simulink model "s_deng_rev1_13_wide"  (R2016b)
(part 3 of 74)

      mask prompts: io_dir "I/O direction"; io_delay "I/O delay"; sample_period "Sample period"; names "Bitfield names [msb...lsb]"; bitwidths "Bitfield widths"; bin_pts "Bitfield binary pts"; arith_types "Bitfield types, ufix=0, fix=1, bool=2"; sim_port "Provide sim input/output?"; show_format "Print format string?"
      mask help: A 32-bit software-accessible register. Can be divided into bitfields of varying widths and types using the fields in the block mask.
      mask init:
      | swreg_init(gcb)
      settings: AttributesFormatString=1input:uf32.0 = 32 bits
      mask TypeOptions io_dir: To Processor | From Processor
      mask Callback io_dir:
      | mask_enables = get_param(gcb, 'MaskEnables');
      | mask_names = get_param(gcb, 'MaskNames');
      | if strcmp(get_param(gcb, 'io_dir'), 'To Processor'),
      |     mask_enables{ismember(mask_names, 'sample_period')} = 'off';
      | else
      |     mask_enables{ismember(mask_names, 'sample_period')} = 'on';
      | end
      | set_param(gcb, 'MaskEnables', mask_enables);
  rpt_length_wng0 : Subsystem  Tag=xps:sw_reg  AncestorBlock=xps_library/software_register  mask(swreg){io_dir=From Processor, io_delay=1, sample_period=1, names=samples, bitwidths=32, bin_pts=0, arith_types=0, sim_port=on, show_format=on}
      mask prompts: io_dir "I/O direction"; io_delay "I/O delay"; sample_period "Sample period"; names "Bitfield names [msb...lsb]"; bitwidths "Bitfield widths"; bin_pts "Bitfield binary pts"; arith_types "Bitfield types, ufix=0, fix=1, bool=2"; sim_port "Provide sim input/output?"; show_format "Print format string?"
      mask help: A 32-bit software-accessible register. Can be divided into bitfields of varying widths and types using the fields in the block mask.
      mask init:
      | swreg_init(gcb)
      settings: AttributesFormatString=1input:uf32.0 = 32 bits
      mask TypeOptions io_dir: To Processor | From Processor
      mask Callback io_dir:
      | mask_enables = get_param(gcb, 'MaskEnables');
      | mask_names = get_param(gcb, 'MaskNames');
      | if strcmp(get_param(gcb, 'io_dir'), 'To Processor'),
      |     mask_enables{ismember(mask_names, 'sample_period')} = 'off';
      | else
      |     mask_enables{ismember(mask_names, 'sample_period')} = 'on';
      | end
      | set_param(gcb, 'MaskEnables', mask_enables);
  rpt_load_time_lsw_wng0 : Subsystem  Tag=xps:sw_reg  AncestorBlock=xps_library/software_register  mask(swreg){io_dir=From Processor, io_delay=1, sample_period=1, names=reg, bitwidths=32, bin_pts=0, arith_types=0, sim_port=on, show_format=on}
      mask prompts: io_dir "I/O direction"; io_delay "I/O delay"; sample_period "Sample period"; names "Bitfield names [msb...lsb]"; bitwidths "Bitfield widths"; bin_pts "Bitfield binary pts"; arith_types "Bitfield types, ufix=0, fix=1, bool=2"; sim_port "Provide sim input/output?"; show_format "Print format string?"
      mask help: A 32-bit software-accessible register. Can be divided into bitfields of varying widths and types using the fields in the block mask.
      mask init:
      | swreg_init(gcb)
      settings: AttributesFormatString=1input:uf32.0 = 32 bits
      mask TypeOptions io_dir: To Processor | From Processor
      mask Callback io_dir:
      | mask_enables = get_param(gcb, 'MaskEnables');
      | mask_names = get_param(gcb, 'MaskNames');
      | if strcmp(get_param(gcb, 'io_dir'), 'To Processor'),
      |     mask_enables{ismember(mask_names, 'sample_period')} = 'off';
      | else
      |     mask_enables{ismember(mask_names, 'sample_period')} = 'on';
      | end
      | set_param(gcb, 'MaskEnables', mask_enables);
  rpt_load_time_msw_wng0 : Subsystem  Tag=xps:sw_reg  AncestorBlock=xps_library/software_register  mask(swreg){io_dir=From Processor, io_delay=1, sample_period=1, names=reg, bitwidths=32, bin_pts=0, arith_types=0, sim_port=on, show_format=on}
      mask prompts: io_dir "I/O direction"; io_delay "I/O delay"; sample_period "Sample period"; names "Bitfield names [msb...lsb]"; bitwidths "Bitfield widths"; bin_pts "Bitfield binary pts"; arith_types "Bitfield types, ufix=0, fix=1, bool=2"; sim_port "Provide sim input/output?"; show_format "Print format string?"
      mask help: A 32-bit software-accessible register. Can be divided into bitfields of varying widths and types using the fields in the block mask.
      mask init:
      | swreg_init(gcb)
      settings: AttributesFormatString=1input:uf32.0 = 32 bits
      mask TypeOptions io_dir: To Processor | From Processor
      mask Callback io_dir:
      | mask_enables = get_param(gcb, 'MaskEnables');
      | mask_names = get_param(gcb, 'MaskNames');
      | if strcmp(get_param(gcb, 'io_dir'), 'To Processor'),
      |     mask_enables{ismember(mask_names, 'sample_period')} = 'off';
      | else
      |     mask_enables{ismember(mask_names, 'sample_period')} = 'on';
      | end
      | set_param(gcb, 'MaskEnables', mask_enables);
  sample_masking : Subsystem  mask{dbwidth=1}
      mask prompts: dbwidth "Data bitwidth:"
  scale_cwg0 : Subsystem  Tag=xps:sw_reg  AncestorBlock=xps_library/software_register  mask(swreg){io_dir=From Processor, io_delay=1, sample_period=1, names=[scale dummy], bitwidths=16, bin_pts=15, arith_types=0, sim_port=on, show_format=on}
      mask prompts: io_dir "I/O direction"; io_delay "I/O delay"; sample_period "Sample period"; names "Bitfield names [msb...lsb]"; bitwidths "Bitfield widths"; bin_pts "Bitfield binary pts"; arith_types "Bitfield types, ufix=0, fix=1, bool=2"; sim_port "Provide sim input/output?"; show_format "Print format string?"
      mask help: A 32-bit software-accessible register. Can be divided into bitfields of varying widths and types using the fields in the block mask.
      mask init:
      | swreg_init(gcb)
      settings: AttributesFormatString=2 inputs:uf16.15,uf16.15 = 32 bits
      mask TypeOptions io_dir: To Processor | From Processor
      mask Callback io_dir:
      | mask_enables = get_param(gcb, 'MaskEnables');
      | mask_names = get_param(gcb, 'MaskNames');
      | if strcmp(get_param(gcb, 'io_dir'), 'To Processor'),
      |     mask_enables{ismember(mask_names, 'sample_period')} = 'off';
      | else
      |     mask_enables{ismember(mask_names, 'sample_period')} = 'on';
      | end
      | set_param(gcb, 'MaskEnables', mask_enables);
  scale_cwg1 : Subsystem  Tag=xps:sw_reg  AncestorBlock=xps_library/software_register  mask(swreg){io_dir=From Processor, io_delay=1, sample_period=1, names=[scale dummy], bitwidths=16, bin_pts=15, arith_types=0, sim_port=on, show_format=on}
      mask prompts: io_dir "I/O direction"; io_delay "I/O delay"; sample_period "Sample period"; names "Bitfield names [msb...lsb]"; bitwidths "Bitfield widths"; bin_pts "Bitfield binary pts"; arith_types "Bitfield types, ufix=0, fix=1, bool=2"; sim_port "Provide sim input/output?"; show_format "Print format string?"
      mask help: A 32-bit software-accessible register. Can be divided into bitfields of varying widths and types using the fields in the block mask.
      mask init:
      | swreg_init(gcb)
      settings: AttributesFormatString=2 inputs:uf16.15,uf16.15 = 32 bits
      mask TypeOptions io_dir: To Processor | From Processor
      mask Callback io_dir:
      | mask_enables = get_param(gcb, 'MaskEnables');
      | mask_names = get_param(gcb, 'MaskNames');
      | if strcmp(get_param(gcb, 'io_dir'), 'To Processor'),
      |     mask_enables{ismember(mask_names, 'sample_period')} = 'off';
      | else
      |     mask_enables{ismember(mask_names, 'sample_period')} = 'on';
      | end
      | set_param(gcb, 'MaskEnables', mask_enables);
  scale_cwg_corr : Subsystem  Tag=xps:sw_reg  AncestorBlock=xps_library/software_register  mask(swreg){io_dir=From Processor, io_delay=1, sample_period=1, names=[scale dummy], bitwidths=16, bin_pts=15, arith_types=0, sim_port=on, show_format=on}
      mask prompts: io_dir "I/O direction"; io_delay "I/O delay"; sample_period "Sample period"; names "Bitfield names [msb...lsb]"; bitwidths "Bitfield widths"; bin_pts "Bitfield binary pts"; arith_types "Bitfield types, ufix=0, fix=1, bool=2"; sim_port "Provide sim input/output?"; show_format "Print format string?"
      mask help: A 32-bit software-accessible register. Can be divided into bitfields of varying widths and types using the fields in the block mask.
      mask init:
      | swreg_init(gcb)
      settings: AttributesFormatString=2 inputs:uf16.15,uf16.15 = 32 bits
      mask TypeOptions io_dir: To Processor | From Processor
      mask Callback io_dir:
      | mask_enables = get_param(gcb, 'MaskEnables');
      | mask_names = get_param(gcb, 'MaskNames');
      | if strcmp(get_param(gcb, 'io_dir'), 'To Processor'),
      |     mask_enables{ismember(mask_names, 'sample_period')} = 'off';
      | else
      |     mask_enables{ismember(mask_names, 'sample_period')} = 'on';
      | end
      | set_param(gcb, 'MaskEnables', mask_enables);
  scale_out0 : Subsystem  Tag=xps:sw_reg  AncestorBlock=xps_library/software_register  mask(swreg){io_dir=From Processor, io_delay=1, sample_period=1, names=[scale dummy], bitwidths=16, bin_pts=15, arith_types=0, sim_port=on, show_format=on}
      mask prompts: io_dir "I/O direction"; io_delay "I/O delay"; sample_period "Sample period"; names "Bitfield names [msb...lsb]"; bitwidths "Bitfield widths"; bin_pts "Bitfield binary pts"; arith_types "Bitfield types, ufix=0, fix=1, bool=2"; sim_port "Provide sim input/output?"; show_format "Print format string?"
      mask help: A 32-bit software-accessible register. Can be divided into bitfields of varying widths and types using the fields in the block mask.
      mask init:
      | swreg_init(gcb)
      settings: AttributesFormatString=2 inputs:uf16.15,uf16.15 = 32 bits
      mask TypeOptions io_dir: To Processor | From Processor
      mask Callback io_dir:
      | mask_enables = get_param(gcb, 'MaskEnables');
      | mask_names = get_param(gcb, 'MaskNames');
      | if strcmp(get_param(gcb, 'io_dir'), 'To Processor'),
      |     mask_enables{ismember(mask_names, 'sample_period')} = 'off';
      | else
      |     mask_enables{ismember(mask_names, 'sample_period')} = 'on';
      | end
      | set_param(gcb, 'MaskEnables', mask_enables);
  scale_out1 : Subsystem  Tag=xps:sw_reg  AncestorBlock=xps_library/software_register  mask(swreg){io_dir=From Processor, io_delay=1, sample_period=1, names=[scale dummy], bitwidths=16, bin_pts=15, arith_types=0, sim_port=on, show_format=on}
      mask prompts: io_dir "I/O direction"; io_delay "I/O delay"; sample_period "Sample period"; names "Bitfield names [msb...lsb]"; bitwidths "Bitfield widths"; bin_pts "Bitfield binary pts"; arith_types "Bitfield types, ufix=0, fix=1, bool=2"; sim_port "Provide sim input/output?"; show_format "Print format string?"
      mask help: A 32-bit software-accessible register. Can be divided into bitfields of varying widths and types using the fields in the block mask.
      mask init:
      | swreg_init(gcb)
      settings: AttributesFormatString=2 inputs:uf16.15,uf16.15 = 32 bits
      mask TypeOptions io_dir: To Processor | From Processor
      mask Callback io_dir:
      | mask_enables = get_param(gcb, 'MaskEnables');
      | mask_names = get_param(gcb, 'MaskNames');
      | if strcmp(get_param(gcb, 'io_dir'), 'To Processor'),
      |     mask_enables{ismember(mask_names, 'sample_period')} = 'off';
      | else
      |     mask_enables{ismember(mask_names, 'sample_period')} = 'on';
      | end
      | set_param(gcb, 'MaskEnables', mask_enables);
  scale_wng0 : Subsystem  Tag=xps:sw_reg  AncestorBlock=xps_library/software_register  mask(swreg){io_dir=From Processor, io_delay=1, sample_period=1, names=[scale dummy], bitwidths=16, bin_pts=15, arith_types=0, sim_port=on, show_format=on}
      mask prompts: io_dir "I/O direction"; io_delay "I/O delay"; sample_period "Sample period"; names "Bitfield names [msb...lsb]"; bitwidths "Bitfield widths"; bin_pts "Bitfield binary pts"; arith_types "Bitfield types, ufix=0, fix=1, bool=2"; sim_port "Provide sim input/output?"; show_format "Print format string?"
      mask help: A 32-bit software-accessible register. Can be divided into bitfields of varying widths and types using the fields in the block mask.
      mask init:
      | swreg_init(gcb)
      settings: AttributesFormatString=2 inputs:uf16.15,uf16.15 = 32 bits
      mask TypeOptions io_dir: To Processor | From Processor
      mask Callback io_dir:
      | mask_enables = get_param(gcb, 'MaskEnables');
      | mask_names = get_param(gcb, 'MaskNames');
      | if strcmp(get_param(gcb, 'io_dir'), 'To Processor'),
      |     mask_enables{ismember(mask_names, 'sample_period')} = 'off';
      | else
      |     mask_enables{ismember(mask_names, 'sample_period')} = 'on';
      | end
      | set_param(gcb, 'MaskEnables', mask_enables);
  scale_wng1 : Subsystem  Tag=xps:sw_reg  AncestorBlock=xps_library/software_register  mask(swreg){io_dir=From Processor, io_delay=1, sample_period=1, names=[scale dummy], bitwidths=16, bin_pts=15, arith_types=0, sim_port=on, show_format=on}
      mask prompts: io_dir "I/O direction"; io_delay "I/O delay"; sample_period "Sample period"; names "Bitfield names [msb...lsb]"; bitwidths "Bitfield widths"; bin_pts "Bitfield binary pts"; arith_types "Bitfield types, ufix=0, fix=1, bool=2"; sim_port "Provide sim input/output?"; show_format "Print format string?"
      mask help: A 32-bit software-accessible register. Can be divided into bitfields of varying widths and types using the fields in the block mask.
      mask init:
      | swreg_init(gcb)
      settings: AttributesFormatString=2 inputs:uf16.15,uf16.15 = 32 bits
      mask TypeOptions io_dir: To Processor | From Processor
      mask Callback io_dir:
      | mask_enables = get_param(gcb, 'MaskEnables');
      | mask_names = get_param(gcb, 'MaskNames');
      | if strcmp(get_param(gcb, 'io_dir'), 'To Processor'),
      |     mask_enables{ismember(mask_names, 'sample_period')} = 'off';
      | else
      |     mask_enables{ismember(mask_names, 'sample_period')} = 'on';
      | end
      | set_param(gcb, 'MaskEnables', mask_enables);
  scale_wng_corr : Subsystem  Tag=xps:sw_reg  AncestorBlock=xps_library/software_register  mask(swreg){io_dir=From Processor, io_delay=1, sample_period=1, names=[scale dummy], bitwidths=16, bin_pts=15, arith_types=0, sim_port=on, show_format=on}
      mask prompts: io_dir "I/O direction"; io_delay "I/O delay"; sample_period "Sample period"; names "Bitfield names [msb...lsb]"; bitwidths "Bitfield widths"; bin_pts "Bitfield binary pts"; arith_types "Bitfield types, ufix=0, fix=1, bool=2"; sim_port "Provide sim input/output?"; show_format "Print format string?"
      mask help: A 32-bit software-accessible register. Can be divided into bitfields of varying widths and types using the fields in the block mask.
      mask init:
      | swreg_init(gcb)
      settings: AttributesFormatString=2 inputs:uf16.15,uf16.15 = 32 bits
      mask TypeOptions io_dir: To Processor | From Processor
      mask Callback io_dir:
      | mask_enables = get_param(gcb, 'MaskEnables');
      | mask_names = get_param(gcb, 'MaskNames');
      | if strcmp(get_param(gcb, 'io_dir'), 'To Processor'),
      |     mask_enables{ismember(mask_names, 'sample_period')} = 'off';
      | else
      |     mask_enables{ismember(mask_names, 'sample_period')} = 'on';
      | end
      | set_param(gcb, 'MaskEnables', mask_enables);
  slice1 : xbsIndex_r4/Slice  nbits=32  boolean_output=off  mode=Lower Bit Location + Width  bit1=-7  base1=MSB of Input  bit0=0  base0=LSB of Input  dbl_ovrd=off  block_type=slice
  slice2 : xbsIndex_r4/Slice  nbits=32  boolean_output=off  mode=Lower Bit Location + Width  bit1=-32  base1=MSB of Input  bit0=32  base0=LSB of Input  dbl_ovrd=off  block_type=slice
  spead_detail : Subsystem  Tag=casper:bitsnap  AncestorBlock=casper_library_scopes/bitfield_snapshot  mask(bitsnap){io_names=[eof we], io_widths=[1 1], io_bps=[0 0], io_types=[2 2], show_format=on, snap_storage=bram, snap_dram_dimm=2, snap_dram_clock=250, snap_nsamples=15, snap_data_width=32, snap_offset=off, snap_circap=off, snap_value=off, snap_ext_arm=off, snap_provide_outputs=on, snap_use_dsp48=on, snap_delay=2, extra_names=[c d], extra_widths=[30 2], extra_bps=[0 0], extra_types=[0 0]}
      mask prompts: io_names "Names [msb...lsb]"; io_widths "Bitwidths [msb...lsb]"; io_bps "Binary pts [msb...lsb]"; io_types "Data types [msb...lsb], ufix=0, fix=1, bool=2"; show_format "Print format string?"; snap_storage "Storage medium"; snap_dram_dimm "DRAM dimm"; snap_dram_clock "DRAM clock rate"; snap_nsamples "Number of Samples (2^?)"; snap_data_width "Data width"; snap_offset "Start delay support"; snap_circap "Circular capture support"; snap_value "Extra value capture support"; snap_ext_arm "External arm support"; snap_provide_outputs "Provide outputs"; snap_use_dsp48 "Use DSP48s to implement counters"; snap_delay "Pre-snapshot delay"; extra_names "Names [msb...lsb]"; extra_widths "Widths [msb...lsb]"; extra_bps "Binary pts [msb...lsb]"; extra_types "Data types [msb...lsb], ufix=0, fix=1, bool=2"
      mask help:
      | A wrapped snapshot block. Allows specification of inputs to a snapblock word so the toolflow can automatically set up the scope.
      | See documentation for snapshot for explanation of parameters.
      mask init:
      | bitsnap_init(gcb);
      settings: AttributesFormatString=|
      | snap(2):b,b = 2 bits\n32 wide, 32768 deep
      | debugID: 29988897
      mask TypeOptions snap_storage: bram | dram
      mask Callback snap_storage: bitsnap_callback();
      mask TypeOptions snap_dram_dimm: 1 | 2 | 3 | 4
      mask TypeOptions snap_dram_clock: 200 | 250 | 266 | 300 | 333
      mask TypeOptions snap_data_width: 8 | 16 | 32 | 64 | 128
      mask Callback snap_value: bitsnap_callback();
      mask Callback snap_ext_arm: bitsnap_callback();
      mask Callback snap_provide_outputs: bitsnap_callback();
  spead_pack0 : Subsystem  Tag=casper:spead_pack  AncestorBlock=casper_library_communications/spead_pack  mask(pkt_pack_mask){max_pkt_len_bits=10, header_ids=0x1600, 0x3101, 0x3102, header_ind_ids=0x3300, spead_msw=64, spead_lsw=48, spead_version=4, bytes_per_word=8}
      mask prompts: max_pkt_len_bits "Max pkt length, 2^? 64-bit words"; header_ids "SPEAD direct address IDs (decimal)"; header_ind_ids "SPEAD indirect address IDs (decimal)"; spead_msw "SPEAD Flavour (MSw)"; spead_lsw "SPEAD Flavour (LSw)"; spead_version "SPEAD version"; bytes_per_word "Word size, in bytes"
      mask help:
      | This block generates SPEAD-compliant packets from a datastream.
      |
      | Packets are created with a fixed header followed by a number of 64-bit items.
      |
      | Requires a 64-bit data stream.
      |
      | The data_ready signal is one cycle BEFORE valid data! Does not have to be with a valid signal either.
      mask init:
      | if floor(log2(bytes_per_word)) ~= log2(bytes_per_word)
      |     error('Bytes per word should be a power of two.');
      | end
      | 
      | spead_pack_init(gcb)
  spead_pack1 : Subsystem  Tag=casper:spead_pack  AncestorBlock=casper_library_communications/spead_pack  mask(pkt_pack_mask){max_pkt_len_bits=10, header_ids=0x1600, 0x3101, 0x3102, header_ind_ids=0x3300, spead_msw=64, spead_lsw=48, spead_version=4, bytes_per_word=8}
      mask prompts: max_pkt_len_bits "Max pkt length, 2^? 64-bit words"; header_ids "SPEAD direct address IDs (decimal)"; header_ind_ids "SPEAD indirect address IDs (decimal)"; spead_msw "SPEAD Flavour (MSw)"; spead_lsw "SPEAD Flavour (LSw)"; spead_version "SPEAD version"; bytes_per_word "Word size, in bytes"
      mask help:
      | This block generates SPEAD-compliant packets from a datastream.
      |
      | Packets are created with a fixed header followed by a number of 64-bit items.
      |
      | Requires a 64-bit data stream.
      |
      | The data_ready signal is one cycle BEFORE valid data! Does not have to be with a valid signal either.
      mask init:
      | if floor(log2(bytes_per_word)) ~= log2(bytes_per_word)
      |     error('Bytes per word should be a power of two.');
      | end
      | 
      | spead_pack_init(gcb)
  spead_pack2 : Subsystem  Tag=casper:spead_pack  AncestorBlock=casper_library_communications/spead_pack  mask(pkt_pack_mask){max_pkt_len_bits=10, header_ids=0x1600, 0x3101, 0x3102, header_ind_ids=0x3300, spead_msw=64, spead_lsw=48, spead_version=4, bytes_per_word=8}
      mask prompts: max_pkt_len_bits "Max pkt length, 2^? 64-bit words"; header_ids "SPEAD direct address IDs (decimal)"; header_ind_ids "SPEAD indirect address IDs (decimal)"; spead_msw "SPEAD Flavour (MSw)"; spead_lsw "SPEAD Flavour (LSw)"; spead_version "SPEAD version"; bytes_per_word "Word size, in bytes"
      mask help:
      | This block generates SPEAD-compliant packets from a datastream.
      |
      | Packets are created with a fixed header followed by a number of 64-bit items.
      |
      | Requires a 64-bit data stream.
      |
      | The data_ready signal is one cycle BEFORE valid data! Does not have to be with a valid signal either.
      mask init:
      | if floor(log2(bytes_per_word)) ~= log2(bytes_per_word)
      |     error('Bytes per word should be a power of two.');
      | end
      | 
      | spead_pack_init(gcb)
  spead_pack3 : Subsystem  Tag=casper:spead_pack  AncestorBlock=casper_library_communications/spead_pack  mask(pkt_pack_mask){max_pkt_len_bits=10, header_ids=0x1600, 0x3101, 0x3102, header_ind_ids=0x3300, spead_msw=64, spead_lsw=48, spead_version=4, bytes_per_word=8}
      mask prompts: max_pkt_len_bits "Max pkt length, 2^? 64-bit words"; header_ids "SPEAD direct address IDs (decimal)"; header_ind_ids "SPEAD indirect address IDs (decimal)"; spead_msw "SPEAD Flavour (MSw)"; spead_lsw "SPEAD Flavour (LSw)"; spead_version "SPEAD version"; bytes_per_word "Word size, in bytes"
      mask help:
      | This block generates SPEAD-compliant packets from a datastream.
      |
      | Packets are created with a fixed header followed by a number of 64-bit items.
      |
      | Requires a 64-bit data stream.
      |
      | The data_ready signal is one cycle BEFORE valid data! Does not have to be with a valid signal either.
      mask init:
      | if floor(log2(bytes_per_word)) ~= log2(bytes_per_word)
      |     error('Bytes per word should be a power of two.');
      | end
      | 
      | spead_pack_init(gcb)
  spead_snap0 : Subsystem  Tag=casper:bitsnap  AncestorBlock=casper_library_scopes/bitfield_snapshot  mask(bitsnap){io_names=[d64], io_widths=64, io_bps=0, io_types=0, show_format=on, snap_storage=bram, snap_dram_dimm=2, snap_dram_clock=250, snap_nsamples=15, snap_data_width=64, snap_offset=off, snap_circap=off, snap_value=off, snap_ext_arm=off, snap_provide_outputs=on, snap_use_dsp48=on, snap_delay=2, extra_names=[c d], extra_widths=[30 2], extra_bps=[0 0], extra_types=[0 0]}
      mask prompts: io_names "Names [msb...lsb]"; io_widths "Bitwidths [msb...lsb]"; io_bps "Binary pts [msb...lsb]"; io_types "Data types [msb...lsb], ufix=0, fix=1, bool=2"; show_format "Print format string?"; snap_storage "Storage medium"; snap_dram_dimm "DRAM dimm"; snap_dram_clock "DRAM clock rate"; snap_nsamples "Number of Samples (2^?)"; snap_data_width "Data width"; snap_offset "Start delay support"; snap_circap "Circular capture support"; snap_value "Extra value capture support"; snap_ext_arm "External arm support"; snap_provide_outputs "Provide outputs"; snap_use_dsp48 "Use DSP48s to implement counters"; snap_delay "Pre-snapshot delay"; extra_names "Names [msb...lsb]"; extra_widths "Widths [msb...lsb]"; extra_bps "Binary pts [msb...lsb]"; extra_types "Data types [msb...lsb], ufix=0, fix=1, bool=2"
      mask help:
      | A wrapped snapshot block. Allows specification of inputs to a snapblock word so the toolflow can automatically set up the scope.
      | See documentation for snapshot for explanation of parameters.
      mask init:
      | bitsnap_init(gcb);
      settings: AttributesFormatString=|
      | snap(1):uf64.0 = 64 bits\n64 wide, 32768 deep
      | debugID: 109311942
      mask TypeOptions snap_storage: bram | dram
      mask Callback snap_storage: bitsnap_callback();
      mask TypeOptions snap_dram_dimm: 1 | 2 | 3 | 4
      mask TypeOptions snap_dram_clock: 200 | 250 | 266 | 300 | 333
      mask TypeOptions snap_data_width: 8 | 16 | 32 | 64 | 128
      mask Callback snap_value: bitsnap_callback();
      mask Callback snap_ext_arm: bitsnap_callback();
      mask Callback snap_provide_outputs: bitsnap_callback();
  speadsnap_control : Subsystem  Tag=xps:sw_reg  AncestorBlock=xps_library/software_register  mask(swreg){io_dir=From Processor, io_delay=0, sample_period=1, names=[speadsnap_arm], bitwidths=1, bin_pts=0, arith_types=2, sim_port=off, show_format=on}
      mask prompts: io_dir "I/O direction"; io_delay "I/O delay"; sample_period "Sample period"; names "Bitfield names [msb...lsb]"; bitwidths "Bitfield widths"; bin_pts "Bitfield binary pts"; arith_types "Bitfield types, ufix=0, fix=1, bool=2"; sim_port "Provide sim input/output?"; show_format "Print format string?"
      mask help: A 32-bit software-accessible register. Can be divided into bitfields of varying widths and types using the fields in the block mask.
      mask init:
      | swreg_init(gcb)
      settings: AttributesFormatString=1input:b = 1 bits
      mask TypeOptions io_dir: To Processor | From Processor
      mask Callback io_dir:
      | mask_enables = get_param(gcb, 'MaskEnables');
      | mask_names = get_param(gcb, 'MaskNames');
      | if strcmp(get_param(gcb, 'io_dir'), 'To Processor'),
      |     mask_enables{ismember(mask_names, 'sample_period')} = 'off';
      | else
      |     mask_enables{ismember(mask_names, 'sample_period')} = 'on';
      | end
      | set_param(gcb, 'MaskEnables', mask_enables);
  speadtime0_offset : Subsystem  Tag=xps:sw_reg  AncestorBlock=xps_library/software_register  mask(swreg){io_dir=From Processor, io_delay=1, sample_period=1, names=speadtime_offset0, bitwidths=32, bin_pts=0, arith_types=0, sim_port=on, show_format=on}
      mask prompts: io_dir "I/O direction"; io_delay "I/O delay"; sample_period "Sample period"; names "Bitfield names [msb...lsb]"; bitwidths "Bitfield widths"; bin_pts "Bitfield binary pts"; arith_types "Bitfield types, ufix=0, fix=1, bool=2"; sim_port "Provide sim input/output?"; show_format "Print format string?"
      mask help: A 32-bit software-accessible register. Can be divided into bitfields of varying widths and types using the fields in the block mask.
      mask init:
      | swreg_init(gcb)
      settings: AttributesFormatString=1input:uf32.0 = 32 bits
      mask TypeOptions io_dir: To Processor | From Processor
      mask Callback io_dir:
      | mask_enables = get_param(gcb, 'MaskEnables');
      | mask_names = get_param(gcb, 'MaskNames');
      | if strcmp(get_param(gcb, 'io_dir'), 'To Processor'),
      |     mask_enables{ismember(mask_names, 'sample_period')} = 'off';
      | else
      |     mask_enables{ismember(mask_names, 'sample_period')} = 'on';
      | end
      | set_param(gcb, 'MaskEnables', mask_enables);
  speadtime1_offset : Subsystem  Tag=xps:sw_reg  AncestorBlock=xps_library/software_register  mask(swreg){io_dir=From Processor, io_delay=1, sample_period=1, names=speadtime_offset1, bitwidths=32, bin_pts=0, arith_types=0, sim_port=on, show_format=on}
      mask prompts: io_dir "I/O direction"; io_delay "I/O delay"; sample_period "Sample period"; names "Bitfield names [msb...lsb]"; bitwidths "Bitfield widths"; bin_pts "Bitfield binary pts"; arith_types "Bitfield types, ufix=0, fix=1, bool=2"; sim_port "Provide sim input/output?"; show_format "Print format string?"
      mask help: A 32-bit software-accessible register. Can be divided into bitfields of varying widths and types using the fields in the block mask.
      mask init:
      | swreg_init(gcb)
      settings: AttributesFormatString=1input:uf32.0 = 32 bits
      mask TypeOptions io_dir: To Processor | From Processor
      mask Callback io_dir:
      | mask_enables = get_param(gcb, 'MaskEnables');
      | mask_names = get_param(gcb, 'MaskNames');
      | if strcmp(get_param(gcb, 'io_dir'), 'To Processor'),
      |     mask_enables{ismember(mask_names, 'sample_period')} = 'off';
      | else
      |     mask_enables{ismember(mask_names, 'sample_period')} = 'on';
      | end
      | set_param(gcb, 'MaskEnables', mask_enables);
  src_sel_cntrl : Subsystem  Tag=xps:sw_reg  AncestorBlock=xps_library/software_register  mask(swreg){io_dir=From Processor, io_delay=1, sample_period=1, names=[src_sel_0 src_sel_1], bitwidths=[2 2], bin_pts=[0 0], arith_types=[0 0], sim_port=on, show_format=on}
      mask prompts: io_dir "I/O direction"; io_delay "I/O delay"; sample_period "Sample period"; names "Bitfield names [msb...lsb]"; bitwidths "Bitfield widths"; bin_pts "Bitfield binary pts"; arith_types "Bitfield types, ufix=0, fix=1, bool=2"; sim_port "Provide sim input/output?"; show_format "Print format string?"
      mask help: A 32-bit software-accessible register. Can be divided into bitfields of varying widths and types using the fields in the block mask.
      mask init:
      | swreg_init(gcb)
      settings: AttributesFormatString=2 inputs:uf2.0,uf2.0 = 4 bits
      mask TypeOptions io_dir: To Processor | From Processor
      mask Callback io_dir:
      | mask_enables = get_param(gcb, 'MaskEnables');
      | mask_names = get_param(gcb, 'MaskNames');
      | if strcmp(get_param(gcb, 'io_dir'), 'To Processor'),
      |     mask_enables{ismember(mask_names, 'sample_period')} = 'off';
      | else
      |     mask_enables{ismember(mask_names, 'sample_period')} = 'on';
      | end
      | set_param(gcb, 'MaskEnables', mask_enables);
  ss_cwg0 : Subsystem  Tag=casper:bitsnap  AncestorBlock=casper_library_scopes/bitfield snapshot  mask(bitsnap){io_names=[d0 d1 d2 d3 d4 d5 d6 d7 gpio_trig], io_widths=[10 10 10 10 10 10 10 10 1], io_bps=[9 9 9 9 9 9 9 9 0], io_types=[1 1 1 1 1 1 1 1 2], show_format=on, snap_storage=bram, snap_dram_dimm=2, snap_dram_clock=250, snap_nsamples=11, snap_data_width=128, snap_offset=on, snap_circap=off, snap_value=off, snap_use_dsp48=off, snap_delay=1, extra_names=[c d], extra_widths=[30 2], extra_bps=[0 0], extra_types=[0 0]}
      mask prompts: io_names "Names [msb...lsb]"; io_widths "Bitwidths [msb...lsb]"; io_bps "Binary pts [msb...lsb]"; io_types "Data types [msb...lsb], ufix=0, fix=1, bool=2"; show_format "Print format string?"; snap_storage "Storage medium"; snap_dram_dimm "DRAM dimm"; snap_dram_clock "DRAM clock rate"; snap_nsamples "Number of Samples (2^?)"; snap_data_width "Data width"; snap_offset "Start delay support"; snap_circap "Circular capture support"; snap_value "Extra value capture support"; snap_use_dsp48 "Use DSP48s to implement counters"; snap_delay "Pre-snapshot delay"; extra_names "Names [msb...lsb]"; extra_widths "Widths [msb...lsb]"; extra_bps "Binary pts [msb...lsb]"; extra_types "Data types [msb...lsb], ufix=0, fix=1, bool=2"
      mask help:
      | A wrapped snapshot block. Allows specification of inputs to a snapblock word so the toolflow can automatically set up the scope.
      | See documentation for snapshot for explanation of parameters.
      mask init:
      | bitsnap_init(gcb);
      settings: AttributesFormatString=|
      | snap(9):f10.9,f10.9,f10.9,f10.9,f10.9,f10.9,f10.9,f10.9,b = 81 bits\n128 wide, 2048 deep
      | debugID: 35994012
      mask TypeOptions snap_storage: bram | dram
      mask Callback snap_storage: bitsnap_callback();
      mask TypeOptions snap_dram_dimm: 1 | 2 | 3 | 4
      mask TypeOptions snap_dram_clock: 200 | 250 | 266 | 300 | 333
      mask TypeOptions snap_data_width: 8 | 16 | 32 | 64 | 128
      mask Callback snap_value: bitsnap_callback();
  ss_cwg1 : Subsystem  Tag=casper:bitsnap  AncestorBlock=casper_library_scopes/bitfield snapshot  mask(bitsnap){io_names=[d0 d1 d2 d3 d4 d5 d6 d7 gpio_trig], io_widths=[10 10 10 10 10 10 10 10 1], io_bps=[9 9 9 9 9 9 9 9 0], io_types=[1 1 1 1 1 1 1 1 2], show_format=on, snap_storage=bram, snap_dram_dimm=2, snap_dram_clock=250, snap_nsamples=11, snap_data_width=128, snap_offset=on, snap_circap=off, snap_value=off, snap_use_dsp48=off, snap_delay=1, extra_names=[c d], extra_widths=[30 2], extra_bps=[0 0], extra_types=[0 0]}
      mask prompts: io_names "Names [msb...lsb]"; io_widths "Bitwidths [msb...lsb]"; io_bps "Binary pts [msb...lsb]"; io_types "Data types [msb...lsb], ufix=0, fix=1, bool=2"; show_format "Print format string?"; snap_storage "Storage medium"; snap_dram_dimm "DRAM dimm"; snap_dram_clock "DRAM clock rate"; snap_nsamples "Number of Samples (2^?)"; snap_data_width "Data width"; snap_offset "Start delay support"; snap_circap "Circular capture support"; snap_value "Extra value capture support"; snap_use_dsp48 "Use DSP48s to implement counters"; snap_delay "Pre-snapshot delay"; extra_names "Names [msb...lsb]"; extra_widths "Widths [msb...lsb]"; extra_bps "Binary pts [msb...lsb]"; extra_types "Data types [msb...lsb], ufix=0, fix=1, bool=2"
      mask help:
      | A wrapped snapshot block. Allows specification of inputs to a snapblock word so the toolflow can automatically set up the scope.
      | See documentation for snapshot for explanation of parameters.
      mask init:
      | bitsnap_init(gcb);
      settings: AttributesFormatString=|
      | snap(9):f10.9,f10.9,f10.9,f10.9,f10.9,f10.9,f10.9,f10.9,b = 81 bits\n128 wide, 2048 deep
      | debugID: 36023803
      mask TypeOptions snap_storage: bram | dram
      mask Callback snap_storage: bitsnap_callback();
      mask TypeOptions snap_dram_dimm: 1 | 2 | 3 | 4
      mask TypeOptions snap_dram_clock: 200 | 250 | 266 | 300 | 333
      mask TypeOptions snap_data_width: 8 | 16 | 32 | 64 | 128
      mask Callback snap_value: bitsnap_callback();
  ss_fifo_in : Subsystem  Tag=casper:bitsnap  AncestorBlock=casper_library_scopes/bitfield snapshot  mask(bitsnap){io_names=[d0 d1 d2 d3 d4 d5 d6 d7 gpio_trig], io_widths=[10 10 10 10 10 10 10 10 1], io_bps=[9 9 9 9 9 9 9 9 0], io_types=[1 1 1 1 1 1 1 1 2], show_format=on, snap_storage=bram, snap_dram_dimm=2, snap_dram_clock=250, snap_nsamples=11, snap_data_width=128, snap_offset=on, snap_circap=off, snap_value=off, snap_use_dsp48=off, snap_delay=1, extra_names=[c d], extra_widths=[30 2], extra_bps=[0 0], extra_types=[0 0]}
      mask prompts: io_names "Names [msb...lsb]"; io_widths "Bitwidths [msb...lsb]"; io_bps "Binary pts [msb...lsb]"; io_types "Data types [msb...lsb], ufix=0, fix=1, bool=2"; show_format "Print format string?"; snap_storage "Storage medium"; snap_dram_dimm "DRAM dimm"; snap_dram_clock "DRAM clock rate"; snap_nsamples "Number of Samples (2^?)"; snap_data_width "Data width"; snap_offset "Start delay support"; snap_circap "Circular capture support"; snap_value "Extra value capture support"; snap_use_dsp48 "Use DSP48s to implement counters"; snap_delay "Pre-snapshot delay"; extra_names "Names [msb...lsb]"; extra_widths "Widths [msb...lsb]"; extra_bps "Binary pts [msb...lsb]"; extra_types "Data types [msb...lsb], ufix=0, fix=1, bool=2"
      mask help:
      | A wrapped snapshot block. Allows specification of inputs to a snapblock word so the toolflow can automatically set up the scope.
      | See documentation for snapshot for explanation of parameters.
      mask init:
      | bitsnap_init(gcb);
      settings: AttributesFormatString=|
      | snap(9):f10.9,f10.9,f10.9,f10.9,f10.9,f10.9,f10.9,f10.9,b = 81 bits\n128 wide, 2048 deep
      | debugID: 19588621
      mask TypeOptions snap_storage: bram | dram
      mask Callback snap_storage: bitsnap_callback();
      mask TypeOptions snap_dram_dimm: 1 | 2 | 3 | 4
      mask TypeOptions snap_dram_clock: 200 | 250 | 266 | 300 | 333
      mask TypeOptions snap_data_width: 8 | 16 | 32 | 64 | 128
      mask Callback snap_value: bitsnap_callback();
  ss_localtime : Subsystem  Tag=casper:bitsnap  AncestorBlock=casper_library_scopes/bitfield snapshot  mask(bitsnap){io_names=time, io_widths=64, io_bps=0, io_types=0, show_format=on, snap_storage=bram, snap_dram_dimm=2, snap_dram_clock=250, snap_nsamples=11, snap_data_width=64, snap_offset=on, snap_circap=off, snap_value=off, snap_use_dsp48=off, snap_delay=1, extra_names=[c d], extra_widths=[30 2], extra_bps=[0 0], extra_types=[0 0]}
      mask prompts: io_names "Names [msb...lsb]"; io_widths "Bitwidths [msb...lsb]"; io_bps "Binary pts [msb...lsb]"; io_types "Data types [msb...lsb], ufix=0, fix=1, bool=2"; show_format "Print format string?"; snap_storage "Storage medium"; snap_dram_dimm "DRAM dimm"; snap_dram_clock "DRAM clock rate"; snap_nsamples "Number of Samples (2^?)"; snap_data_width "Data width"; snap_offset "Start delay support"; snap_circap "Circular capture support"; snap_value "Extra value capture support"; snap_use_dsp48 "Use DSP48s to implement counters"; snap_delay "Pre-snapshot delay"; extra_names "Names [msb...lsb]"; extra_widths "Widths [msb...lsb]"; extra_bps "Binary pts [msb...lsb]"; extra_types "Data types [msb...lsb], ufix=0, fix=1, bool=2"
      mask help:
      | A wrapped snapshot block. Allows specification of inputs to a snapblock word so the toolflow can automatically set up the scope.
      | See documentation for snapshot for explanation of parameters.
      mask init:
      | bitsnap_init(gcb);
      settings: AttributesFormatString=|
      | snap(1):uf64.0 = 64 bits\n64 wide, 2048 deep
      | debugID: 69418317
      mask TypeOptions snap_storage: bram | dram
      mask Callback snap_storage: bitsnap_callback();
      mask TypeOptions snap_dram_dimm: 1 | 2 | 3 | 4
      mask TypeOptions snap_dram_clock: 200 | 250 | 266 | 300 | 333
      mask TypeOptions snap_data_width: 8 | 16 | 32 | 64 | 128
      mask Callback snap_value: bitsnap_callback();
  ss_trig_time_lsw : Subsystem  Tag=xps:sw_reg  AncestorBlock=xps_library/software_register  mask(swreg){io_dir=From Processor, io_delay=1, sample_period=1, names=reg, bitwidths=32, bin_pts=0, arith_types=0, sim_port=on, show_format=on}
      mask prompts: io_dir "I/O direction"; io_delay "I/O delay"; sample_period "Sample period"; names "Bitfield names [msb...lsb]"; bitwidths "Bitfield widths"; bin_pts "Bitfield binary pts"; arith_types "Bitfield types, ufix=0, fix=1, bool=2"; sim_port "Provide sim input/output?"; show_format "Print format string?"
      mask help: A 32-bit software-accessible register. Can be divided into bitfields of varying widths and types using the fields in the block mask.
      mask init:
      | swreg_init(gcb)
      settings: AttributesFormatString=1input:uf32.0 = 32 bits
      mask TypeOptions io_dir: To Processor | From Processor
      mask Callback io_dir:
      | mask_enables = get_param(gcb, 'MaskEnables');
      | mask_names = get_param(gcb, 'MaskNames');
      | if strcmp(get_param(gcb, 'io_dir'), 'To Processor'),
      |     mask_enables{ismember(mask_names, 'sample_period')} = 'off';
      | else
      |     mask_enables{ismember(mask_names, 'sample_period')} = 'on';
      | end
      | set_param(gcb, 'MaskEnables', mask_enables);
  ss_trig_time_msw : Subsystem  Tag=xps:sw_reg  AncestorBlock=xps_library/software_register  mask(swreg){io_dir=From Processor, io_delay=1, sample_period=1, names=reg, bitwidths=32, bin_pts=0, arith_types=0, sim_port=on, show_format=on}
      mask prompts: io_dir "I/O direction"; io_delay "I/O delay"; sample_period "Sample period"; names "Bitfield names [msb...lsb]"; bitwidths "Bitfield widths"; bin_pts "Bitfield binary pts"; arith_types "Bitfield types, ufix=0, fix=1, bool=2"; sim_port "Provide sim input/output?"; show_format "Print format string?"
      mask help: A 32-bit software-accessible register. Can be divided into bitfields of varying widths and types using the fields in the block mask.
      mask init:
      | swreg_init(gcb)
      settings: AttributesFormatString=1input:uf32.0 = 32 bits
      mask TypeOptions io_dir: To Processor | From Processor
      mask Callback io_dir:
      | mask_enables = get_param(gcb, 'MaskEnables');
      | mask_names = get_param(gcb, 'MaskNames');
      | if strcmp(get_param(gcb, 'io_dir'), 'To Processor'),
      |     mask_enables{ismember(mask_names, 'sample_period')} = 'off';
      | else
      |     mask_enables{ismember(mask_names, 'sample_period')} = 'on';
      | end
      | set_param(gcb, 'MaskEnables', mask_enables);
  start_flag_lsw : Subsystem  Tag=xps:sw_reg  AncestorBlock=xps_library/software_register  mask(swreg){io_dir=From Processor, io_delay=1, sample_period=1, names=reg, bitwidths=32, bin_pts=0, arith_types=0, sim_port=on, show_format=on}
      mask prompts: io_dir "I/O direction"; io_delay "I/O delay"; sample_period "Sample period"; names "Bitfield names [msb...lsb]"; bitwidths "Bitfield widths"; bin_pts "Bitfield binary pts"; arith_types "Bitfield types, ufix=0, fix=1, bool=2"; sim_port "Provide sim input/output?"; show_format "Print format string?"
      mask help: A 32-bit software-accessible register. Can be divided into bitfields of varying widths and types using the fields in the block mask.
      mask init:
      | swreg_init(gcb)
      settings: AttributesFormatString=1input:uf32.0 = 32 bits
      mask TypeOptions io_dir: To Processor | From Processor
      mask Callback io_dir:
      | mask_enables = get_param(gcb, 'MaskEnables');
      | mask_names = get_param(gcb, 'MaskNames');
      | if strcmp(get_param(gcb, 'io_dir'), 'To Processor'),
      |     mask_enables{ismember(mask_names, 'sample_period')} = 'off';
      | else
      |     mask_enables{ismember(mask_names, 'sample_period')} = 'on';
      | end
      | set_param(gcb, 'MaskEnables', mask_enables);
  start_flag_msw : Subsystem  Tag=xps:sw_reg  AncestorBlock=xps_library/software_register  mask(swreg){io_dir=From Processor, io_delay=1, sample_period=1, names=reg, bitwidths=32, bin_pts=0, arith_types=0, sim_port=on, show_format=on}
      mask prompts: io_dir "I/O direction"; io_delay "I/O delay"; sample_period "Sample period"; names "Bitfield names [msb...lsb]"; bitwidths "Bitfield widths"; bin_pts "Bitfield binary pts"; arith_types "Bitfield types, ufix=0, fix=1, bool=2"; sim_port "Provide sim input/output?"; show_format "Print format string?"
      mask help: A 32-bit software-accessible register. Can be divided into bitfields of varying widths and types using the fields in the block mask.
      mask init:
      | swreg_init(gcb)
      settings: AttributesFormatString=1input:uf32.0 = 32 bits
      mask TypeOptions io_dir: To Processor | From Processor
      mask Callback io_dir:
      | mask_enables = get_param(gcb, 'MaskEnables');
      | mask_names = get_param(gcb, 'MaskNames');
      | if strcmp(get_param(gcb, 'io_dir'), 'To Processor'),
      |     mask_enables{ismember(mask_names, 'sample_period')} = 'off';
      | else
      |     mask_enables{ismember(mask_names, 'sample_period')} = 'on';
      | end
      | set_param(gcb, 'MaskEnables', mask_enables);
  start_load_time_lsw : Subsystem  Tag=xps:sw_reg  AncestorBlock=xps_library/software_register  mask(swreg){io_dir=From Processor, io_delay=1, sample_period=1, names=reg, bitwidths=32, bin_pts=0, arith_types=0, sim_port=on, show_format=on}
      mask prompts: io_dir "I/O direction"; io_delay "I/O delay"; sample_period "Sample period"; names "Bitfield names [msb...lsb]"; bitwidths "Bitfield widths"; bin_pts "Bitfield binary pts"; arith_types "Bitfield types, ufix=0, fix=1, bool=2"; sim_port "Provide sim input/output?"; show_format "Print format string?"
      mask help: A 32-bit software-accessible register. Can be divided into bitfields of varying widths and types using the fields in the block mask.
      mask init:
      | swreg_init(gcb)
      settings: AttributesFormatString=1input:uf32.0 = 32 bits
      mask TypeOptions io_dir: To Processor | From Processor
      mask Callback io_dir:
      | mask_enables = get_param(gcb, 'MaskEnables');
      | mask_names = get_param(gcb, 'MaskNames');
      | if strcmp(get_param(gcb, 'io_dir'), 'To Processor'),
      |     mask_enables{ismember(mask_names, 'sample_period')} = 'off';
      | else
      |     mask_enables{ismember(mask_names, 'sample_period')} = 'on';
      | end
      | set_param(gcb, 'MaskEnables', mask_enables);
  start_load_time_msw : Subsystem  Tag=xps:sw_reg  AncestorBlock=xps_library/software_register  mask(swreg){io_dir=From Processor, io_delay=1, sample_period=1, names=reg, bitwidths=32, bin_pts=0, arith_types=0, sim_port=on, show_format=on}
      mask prompts: io_dir "I/O direction"; io_delay "I/O delay"; sample_period "Sample period"; names "Bitfield names [msb...lsb]"; bitwidths "Bitfield widths"; bin_pts "Bitfield binary pts"; arith_types "Bitfield types, ufix=0, fix=1, bool=2"; sim_port "Provide sim input/output?"; show_format "Print format string?"
      mask help: A 32-bit software-accessible register. Can be divided into bitfields of varying widths and types using the fields in the block mask.
      mask init:
      | swreg_init(gcb)
      settings: AttributesFormatString=1input:uf32.0 = 32 bits
      mask TypeOptions io_dir: To Processor | From Processor
      mask Callback io_dir:
      | mask_enables = get_param(gcb, 'MaskEnables');
      | mask_names = get_param(gcb, 'MaskNames');
      | if strcmp(get_param(gcb, 'io_dir'), 'To Processor'),
      |     mask_enables{ismember(mask_names, 'sample_period')} = 'off';
      | else
      |     mask_enables{ismember(mask_names, 'sample_period')} = 'on';
      | end
      | set_param(gcb, 'MaskEnables', mask_enables);
  start_time_lsw : Subsystem  Tag=xps:sw_reg  AncestorBlock=xps_library/software_register  mask(swreg){io_dir=From Processor, io_delay=1, sample_period=1, names=reg, bitwidths=32, bin_pts=0, arith_types=0, sim_port=on, show_format=on}
      mask prompts: io_dir "I/O direction"; io_delay "I/O delay"; sample_period "Sample period"; names "Bitfield names [msb...lsb]"; bitwidths "Bitfield widths"; bin_pts "Bitfield binary pts"; arith_types "Bitfield types, ufix=0, fix=1, bool=2"; sim_port "Provide sim input/output?"; show_format "Print format string?"
      mask help: A 32-bit software-accessible register. Can be divided into bitfields of varying widths and types using the fields in the block mask.
      mask init:
      | swreg_init(gcb)
      settings: AttributesFormatString=1input:uf32.0 = 32 bits
      mask TypeOptions io_dir: To Processor | From Processor
      mask Callback io_dir:
      | mask_enables = get_param(gcb, 'MaskEnables');
      | mask_names = get_param(gcb, 'MaskNames');
      | if strcmp(get_param(gcb, 'io_dir'), 'To Processor'),
      |     mask_enables{ismember(mask_names, 'sample_period')} = 'off';
      | else
      |     mask_enables{ismember(mask_names, 'sample_period')} = 'on';
      | end
      | set_param(gcb, 'MaskEnables', mask_enables);
  start_time_msw : Subsystem  Tag=xps:sw_reg  AncestorBlock=xps_library/software_register  mask(swreg){io_dir=From Processor, io_delay=1, sample_period=1, names=reg, bitwidths=32, bin_pts=0, arith_types=0, sim_port=on, show_format=on}
      mask prompts: io_dir "I/O direction"; io_delay "I/O delay"; sample_period "Sample period"; names "Bitfield names [msb...lsb]"; bitwidths "Bitfield widths"; bin_pts "Bitfield binary pts"; arith_types "Bitfield types, ufix=0, fix=1, bool=2"; sim_port "Provide sim input/output?"; show_format "Print format string?"
      mask help: A 32-bit software-accessible register. Can be divided into bitfields of varying widths and types using the fields in the block mask.
      mask init:
      | swreg_init(gcb)
      settings: AttributesFormatString=1input:uf32.0 = 32 bits
      mask TypeOptions io_dir: To Processor | From Processor
      mask Callback io_dir:
      | mask_enables = get_param(gcb, 'MaskEnables');
      | mask_names = get_param(gcb, 'MaskNames');
      | if strcmp(get_param(gcb, 'io_dir'), 'To Processor'),
      |     mask_enables{ismember(mask_names, 'sample_period')} = 'off';
      | else
      |     mask_enables{ismember(mask_names, 'sample_period')} = 'on';
      | end
      | set_param(gcb, 'MaskEnables', mask_enables);
  status0 : Subsystem  Tag=xps:sw_reg  AncestorBlock=xps_library/software_register  mask(swreg){io_dir=To Processor, io_delay=0, sample_period=1, names=[led_up led_rx led_tx tx_afull tx_overflow rx_overrun], bitwidths=1, bin_pts=0, arith_types=2, sim_port=off, show_format=on}
      mask prompts: io_dir "I/O direction"; io_delay "I/O delay"; sample_period "Sample period"; names "Bitfield names [msb...lsb]"; bitwidths "Bitfield widths"; bin_pts "Bitfield binary pts"; arith_types "Bitfield types, ufix=0, fix=1, bool=2"; sim_port "Provide sim input/output?"; show_format "Print format string?"
      mask help: A 32-bit software-accessible register. Can be divided into bitfields of varying widths and types using the fields in the block mask.
      mask init:
      | swreg_init(gcb)
      settings: AttributesFormatString=6 outputs:b,b,b,b,b,b = 6 bits
      mask TypeOptions io_dir: To Processor | From Processor
      mask Callback io_dir:
      | mask_enables = get_param(gcb, 'MaskEnables');
      | mask_names = get_param(gcb, 'MaskNames');
      | if strcmp(get_param(gcb, 'io_dir'), 'To Processor'),
      |     mask_enables{ismember(mask_names, 'sample_period')} = 'off';
      | else
      |     mask_enables{ismember(mask_names, 'sample_period')} = 'on';
      | end
      | set_param(gcb, 'MaskEnables', mask_enables);
  stop_load_time_lsw : Subsystem  Tag=xps:sw_reg  AncestorBlock=xps_library/software_register  mask(swreg){io_dir=From Processor, io_delay=1, sample_period=1, names=reg, bitwidths=32, bin_pts=0, arith_types=0, sim_port=on, show_format=on}
      mask prompts: io_dir "I/O direction"; io_delay "I/O delay"; sample_period "Sample period"; names "Bitfield names [msb...lsb]"; bitwidths "Bitfield widths"; bin_pts "Bitfield binary pts"; arith_types "Bitfield types, ufix=0, fix=1, bool=2"; sim_port "Provide sim input/output?"; show_format "Print format string?"
      mask help: A 32-bit software-accessible register. Can be divided into bitfields of varying widths and types using the fields in the block mask.
      mask init:
      | swreg_init(gcb)
      settings: AttributesFormatString=1input:uf32.0 = 32 bits
      mask TypeOptions io_dir: To Processor | From Processor
      mask Callback io_dir:
      | mask_enables = get_param(gcb, 'MaskEnables');
      | mask_names = get_param(gcb, 'MaskNames');
      | if strcmp(get_param(gcb, 'io_dir'), 'To Processor'),
      |     mask_enables{ismember(mask_names, 'sample_period')} = 'off';
      | else
      |     mask_enables{ismember(mask_names, 'sample_period')} = 'on';
      | end
      | set_param(gcb, 'MaskEnables', mask_enables);
  stop_load_time_msw : Subsystem  Tag=xps:sw_reg  AncestorBlock=xps_library/software_register  mask(swreg){io_dir=From Processor, io_delay=1, sample_period=1, names=reg, bitwidths=32, bin_pts=0, arith_types=0, sim_port=on, show_format=on}
      mask prompts: io_dir "I/O direction"; io_delay "I/O delay"; sample_period "Sample period"; names "Bitfield names [msb...lsb]"; bitwidths "Bitfield widths"; bin_pts "Bitfield binary pts"; arith_types "Bitfield types, ufix=0, fix=1, bool=2"; sim_port "Provide sim input/output?"; show_format "Print format string?"
      mask help: A 32-bit software-accessible register. Can be divided into bitfields of varying widths and types using the fields in the block mask.
      mask init:
      | swreg_init(gcb)
      settings: AttributesFormatString=1input:uf32.0 = 32 bits
      mask TypeOptions io_dir: To Processor | From Processor
      mask Callback io_dir:
      | mask_enables = get_param(gcb, 'MaskEnables');
      | mask_names = get_param(gcb, 'MaskNames');
      | if strcmp(get_param(gcb, 'io_dir'), 'To Processor'),
      |     mask_enables{ismember(mask_names, 'sample_period')} = 'off';
      | else
      |     mask_enables{ismember(mask_names, 'sample_period')} = 'on';
      | end
      | set_param(gcb, 'MaskEnables', mask_enables);
  test_control : Subsystem  Tag=xps:sw_reg  AncestorBlock=xps_library/software_register  mask(swreg){io_dir=From Processor, io_delay=0, sample_period=1, names=[sel_ramp80 rst_ramp80], bitwidths=1, bin_pts=0, arith_types=2, sim_port=on, show_format=on}
      mask prompts: io_dir "I/O direction"; io_delay "I/O delay"; sample_period "Sample period"; names "Bitfield names [msb...lsb]"; bitwidths "Bitfield widths"; bin_pts "Bitfield binary pts"; arith_types "Bitfield types, ufix=0, fix=1, bool=2"; sim_port "Provide sim input/output?"; show_format "Print format string?"
      mask help: A 32-bit software-accessible register. Can be divided into bitfields of varying widths and types using the fields in the block mask.
      mask init:
      | swreg_init(gcb)
      settings: AttributesFormatString=2 inputs:b,b = 2 bits
      mask TypeOptions io_dir: To Processor | From Processor
      mask Callback io_dir:
      | mask_enables = get_param(gcb, 'MaskEnables');
      | mask_names = get_param(gcb, 'MaskNames');
      | if strcmp(get_param(gcb, 'io_dir'), 'To Processor'),
      |     mask_enables{ismember(mask_names, 'sample_period')} = 'off';
      | else
      |     mask_enables{ismember(mask_names, 'sample_period')} = 'on';
      | end
      | set_param(gcb, 'MaskEnables', mask_enables);
  tick_offset_lsw : Subsystem  Tag=xps:sw_reg  AncestorBlock=xps_library/software_register  mask(swreg){io_dir=From Processor, io_delay=1, sample_period=1, names=reg, bitwidths=32, bin_pts=0, arith_types=0, sim_port=on, show_format=on}
      mask prompts: io_dir "I/O direction"; io_delay "I/O delay"; sample_period "Sample period"; names "Bitfield names [msb...lsb]"; bitwidths "Bitfield widths"; bin_pts "Bitfield binary pts"; arith_types "Bitfield types, ufix=0, fix=1, bool=2"; sim_port "Provide sim input/output?"; show_format "Print format string?"
      mask help: A 32-bit software-accessible register. Can be divided into bitfields of varying widths and types using the fields in the block mask.
      mask init:
      | swreg_init(gcb)
      settings: AttributesFormatString=1input:uf32.0 = 32 bits
      mask TypeOptions io_dir: To Processor | From Processor
      mask Callback io_dir:
      | mask_enables = get_param(gcb, 'MaskEnables');
      | mask_names = get_param(gcb, 'MaskNames');
      | if strcmp(get_param(gcb, 'io_dir'), 'To Processor'),
      |     mask_enables{ismember(mask_names, 'sample_period')} = 'off';
      | else
      |     mask_enables{ismember(mask_names, 'sample_period')} = 'on';
      | end
      | set_param(gcb, 'MaskEnables', mask_enables);
  tick_offset_msw : Subsystem  Tag=xps:sw_reg  AncestorBlock=xps_library/software_register  mask(swreg){io_dir=From Processor, io_delay=1, sample_period=1, names=reg, bitwidths=32, bin_pts=0, arith_types=0, sim_port=on, show_format=on}
      mask prompts: io_dir "I/O direction"; io_delay "I/O delay"; sample_period "Sample period"; names "Bitfield names [msb...lsb]"; bitwidths "Bitfield widths"; bin_pts "Bitfield binary pts"; arith_types "Bitfield types, ufix=0, fix=1, bool=2"; sim_port "Provide sim input/output?"; show_format "Print format string?"
      mask help: A 32-bit software-accessible register. Can be divided into bitfields of varying widths and types using the fields in the block mask.
      mask init:
      | swreg_init(gcb)
      settings: AttributesFormatString=1input:uf32.0 = 32 bits
      mask TypeOptions io_dir: To Processor | From Processor
      mask Callback io_dir:
      | mask_enables = get_param(gcb, 'MaskEnables');
      | mask_names = get_param(gcb, 'MaskNames');
      | if strcmp(get_param(gcb, 'io_dir'), 'To Processor'),
      |     mask_enables{ismember(mask_names, 'sample_period')} = 'off';
      | else
      |     mask_enables{ismember(mask_names, 'sample_period')} = 'on';
      | end
      | set_param(gcb, 'MaskEnables', mask_enables);
  ticks_since_mrst : Subsystem
  tvg_spead_time_with_pkt_ctr : Subsystem  mask{packetlen_bits=9}
      mask prompts: packetlen_bits "Packet length, num 80-bit words (2^?):"
  tx_afull_cntr : Subsystem  Tag=xps:sw_reg  AncestorBlock=xps_library/software_register  mask(swreg){io_dir=To Processor, io_delay=0, sample_period=1, names=reg, bitwidths=32, bin_pts=0, arith_types=0, sim_port=off, show_format=on}
      mask prompts: io_dir "I/O direction"; io_delay "I/O delay"; sample_period "Sample period"; names "Bitfield names [msb...lsb]"; bitwidths "Bitfield widths"; bin_pts "Bitfield binary pts"; arith_types "Bitfield types, ufix=0, fix=1, bool=2"; sim_port "Provide sim input/output?"; show_format "Print format string?"
      mask help: A 32-bit software-accessible register. Can be divided into bitfields of varying widths and types using the fields in the block mask.
      mask init:
      | swreg_init(gcb)
      settings: AttributesFormatString=1output:uf32.0 = 32 bits
      mask TypeOptions io_dir: To Processor | From Processor
      mask Callback io_dir:
      | mask_enables = get_param(gcb, 'MaskEnables');
      | mask_names = get_param(gcb, 'MaskNames');
      | if strcmp(get_param(gcb, 'io_dir'), 'To Processor'),
      |     mask_enables{ismember(mask_names, 'sample_period')} = 'off';
      | else
      |     mask_enables{ismember(mask_names, 'sample_period')} = 'on';
      | end
      | set_param(gcb, 'MaskEnables', mask_enables);
  tx_of_cntr : Subsystem  Tag=xps:sw_reg  AncestorBlock=xps_library/software_register  mask(swreg){io_dir=To Processor, io_delay=0, sample_period=1, names=reg, bitwidths=32, bin_pts=0, arith_types=0, sim_port=off, show_format=on}
      mask prompts: io_dir "I/O direction"; io_delay "I/O delay"; sample_period "Sample period"; names "Bitfield names [msb...lsb]"; bitwidths "Bitfield widths"; bin_pts "Bitfield binary pts"; arith_types "Bitfield types, ufix=0, fix=1, bool=2"; sim_port "Provide sim input/output?"; show_format "Print format string?"
      mask help: A 32-bit software-accessible register. Can be divided into bitfields of varying widths and types using the fields in the block mask.
      mask init:
      | swreg_init(gcb)
      settings: AttributesFormatString=1output:uf32.0 = 32 bits
      mask TypeOptions io_dir: To Processor | From Processor
      mask Callback io_dir:
      | mask_enables = get_param(gcb, 'MaskEnables');
      | mask_names = get_param(gcb, 'MaskNames');
      | if strcmp(get_param(gcb, 'io_dir'), 'To Processor'),
      |     mask_enables{ismember(mask_names, 'sample_period')} = 'off';
      | else
      |     mask_enables{ismember(mask_names, 'sample_period')} = 'on';
      | end
      | set_param(gcb, 'MaskEnables', mask_enables);
  wng0 : Subsystem
  wng1 : Subsystem
  wng_corr : Subsystem
  wng_rst : Subsystem
  wr_addr{0..3} (4 alike) : xbsIndex_r4/Counter  cnt_type=Free Running  cnt_to=Inf  operation=Up  start_count=0  cnt_by_val=1  arith_type=Unsigned  n_bits=10  bin_pt=0  load_pin=off  rst=on  en=on  explicit_period=on  period=1  use_behavioral_HDL=off  implementation=Fabric  dbl_ovrd=off  block_type=counter
  tag scope: arb_en0=global, arb_rst0=global, dram_addr_offset0=global, dram_rd_repeat0=global, dram_rd_repeat_delay0=global, dram_rd_trig0=global, dram_read_length0=global, dram_tvg0=global, dram_tvg_length0=global, local_time=global, tvg_sel0=global
  wires:
  gbe_porttx/1(in_reg) -> pipeline15/1(d)
  Constant9/1 -> gbe_porttx/1(sim_1)
  Constant10/1 -> gbe_iptx0/1(sim_1)
  Constant12/1 -> gbe_iptx1/1(sim_1)
  Constant13/1 -> gbe_iptx2/1(sim_1)
  Constant14/1 -> gbe_iptx3/1(sim_1)
  Constant15/1 -> digitiser_id/1(sim_1)
  Constant17/1 -> receptor_id/1(sim_1)
  Constant16/1 -> digitiser_id/2(sim_2)
  receptor_id/1(in_receptor_id) -> bus_create/3(in3)
  Constant6/1 -> receptor_id/2(sim_2)
  Constant19/1 -> receptor_id/3(sim_3)
  [masked_time] -> Delay128/1
  tvg_spead_time_with_pkt_ctr/1(local_time) -> Delay131/1
  tvg_spead_time_with_pkt_ctr/3(tvg_data_pol0) -> Delay133/1
  tvg_spead_time_with_pkt_ctr/4(tvg_data_pol1) -> Delay134/1
  tvg_spead_time_with_pkt_ctr/2(spead_time) -> Delay132/1
  [fifoselect] -> edge_detect5/1(in), Inverter2/1
  Register5/1 -> [speadtime0]  "speadtime0"
  Inverter2/1 -> edge_detect6/1(in)
  edge_detect5/1(out) -> Register5/2
  edge_detect6/1(out) -> Register6/2
  Register6/1 -> [speadtime1]  "speadtime1"
  [mrst] -> ticks_since_mrst/1(reset)
  [sync] -> ticks_since_mrst/2(sync)
  ticks_since_mrst/1(time64) -> [local_time]  "localtime"
  [msync] -> [sync]  "sync"
  edge_detect2/1(out) -> [mrst]  "mrst"
  edge_detect1/1(out) -> [msync]  "msync"
  edge_detect4/1(out) -> Terminator81/1  "clr_status"
  [local_time] -> slice1/1, slice2/1
  Constant28/1 -> orig_control/3(sim_3)
  Constant44/1 -> orig_control/1(sim_1)
  Constant24/1 -> orig_control/2(sim_2)
  Constant33/1 -> orig_control/6(sim_6)
  Constant30/1 -> orig_control/5(sim_5)
  Constant36/1 -> orig_control/4(sim_4)
  Pulse Generator/1 -> orig_control/8(sim_8)
  [tick_offset] -> ticks_since_mrst/3(offset)
  edge_detect10/1(out) -> [load_tick_offset]  "mrst"
  Constant20/1 -> orig_control/9(sim_9)
  digitiser_id/1(in_digitiser_serial) -> bus_create/1(in1)
  digitiser_id/2(in_digitiser_type) -> bus_create/2(in2)
  Constant43/1 -> flag_setup/3(sim_3)
  Constant42/1 -> flag_setup/2(sim_2)
  Constant39/1 -> flag_setup/1(sim_1)
  Counter Free-Running3/1 -> Relational Operator4/2
  Constant48/1 -> Relational Operator4/1
  Relational Operator4/1 -> flag_setup/4(sim_4)
  Constant52/1 -> start_flag_msw/1(sim_1)
  Constant53/1 -> start_flag_lsw/1(sim_1)
  Constant51/1 -> end_flag_msw/1(sim_1)
  Constant50/1 -> end_flag_lsw/1(sim_1)
  Concat4/1 -> Delay49/1  "starttime"
  Concat5/1 -> Delay50/1  "stoptime"
  [flag_start_time] -> Delay46/1
  [local_time] -> Delay45/1, Delay47/1
  [flag_end_time] -> Delay48/1, Delay51/1
  Relational/1 -> Logical2/2  "start_okay"
  [flag_armed] -> Delay44/1
  Relational1/1 -> Logical4/2  "end_okay"
  Logical2/1 -> Delay23/1  "start_okay"
  Logical4/1 -> Logical3/1  "end_okay"
  edge_detect9/1(out) -> [load_flag_time]  "loadtimes"
  Constant4/1 -> Register1/1
  edge_detect8/1(out) -> [reset_flag_time]  "rst"
  [reset_flag_time] -> Register1/2
  [load_flag_time] -> Register1/3
  Register1/1 -> [flag_armed]  "armed"
  Relational Operator3/1 -> flag_setup/5(sim_5)
  Relational2/1 -> Delay22/1  "zero_stop"
  Constant2/1 -> Relational2/2
  Logical3/1 -> Logical1/2  "eokay"
  Counter Free-Running2/1 -> Relational Operator3/2
  Constant5/1 -> Relational Operator3/1
  Logical5/1 -> sample_masking/2(den_in)
  Constant49/1 -> start_time_msw/1(sim_1)
  Constant54/1 -> start_time_lsw/1(sim_1)
  Constant3/1 -> end_time_msw/1(sim_1)
  Constant11/1 -> end_time_lsw/1(sim_1)
  Relational3/1 -> Logical6/2  "start_okay"
  Relational4/1 -> Logical8/2  "end_okay"
  [start_time] -> Delay39/1
  Relational6/1 -> Delay15/1  "first_sample"
  [end_time] -> Delay41/1
  Relational7/1 -> Delay16/1  "last_sample"
  [sample_end] -> sample_masking/6(sample_end)
  [sample_start] -> sample_masking/5(sample_start)
  sample_masking/2(den_out) -> Delay126/1  "enable"
  sample_masking/3(data_mask) -> Delay127/1  "mask"
  edge_detect11/1(out) -> [reset_en_time]  "reset_en_time"
  Relational Operator5/1 -> control_output/2(sim_2)
  Counter Free-Running4/1 -> Relational Operator6/2, Relational Operator5/2
  Constant38/1 -> Relational Operator5/1
  edge_detect12/1(out) -> [load_en_time]  "load_en_time"
  Concat/1 -> Delay42/1
  Concat1/1 -> Delay43/1
  Constant22/1 -> Register2/1
  [reset_en_time] -> Register2/2
  [load_en_time] -> Register2/3
  Register2/1 -> [en_armed]  "armed"
  Logical6/1 -> Delay17/1  "start_okay"
  Logical8/1 -> Logical7/1  "end_okay"
  Logical7/1 -> Logical5/2
  Constant34/1 -> Delay37/1
  Relational5/1 -> Delay14/1
  Constant29/1 -> control_output/3(sim_3)
  Constant47/1 -> control_output/4(sim_4)
  Constant31/1 -> Relational Operator6/1
  Relational Operator6/1 -> control_output/1(sim_1)
  [data_enable] -> Delay129/1
  [sample_mask] -> Delay130/1
  Constant46/1 -> tick_offset_msw/1(sim_1)
  Constant7/1 -> tick_offset_lsw/1(sim_1)
  Concat2/1 -> Register3/1
  [load_tick_offset] -> Register3/2
  Register3/1 -> [tick_offset]
  wng0/1(bus_out) -> [wng0_tp0], pipeline78/1(d)
  cwg_corr/1(bus_out) -> pipeline91/1(d), pipeline92/1(d), [Bus_expand_cwg_corr]
  bus_addsub/1(dout) -> Delay105/1
  bus_addsub2/1(dout) -> Delay6/1
  bus_addsub3/1(dout) -> Delay9/1
  bus_addsub1/1(dout) -> Delay5/1
  bus_addsub4/1(dout) -> bus_convert6/1(din)
  bus_mult/1(a*b) -> [cwg0_tp1], bus_convert/1(din)
  bus_addsub5/1(dout) -> bus_convert7/1(din)
  bus_mult1/1(a*b) -> bus_convert1/1(din), [cwg1_tp1]
  scale_out1/1(in_scale) -> Gateway Out3/1, pipeline52/1(d)
  Constant35/1 -> scale_wng0/1(sim_1)
  Constant1/1 -> scale_wng_corr/1(sim_1)
  pipeline21/1(q) -> edge_detect12/1(in)
  pipeline22/1(q) -> edge_detect11/1(in)
  pipeline23/1(q) -> [sample_start]
  pipeline24/1(q) -> [sample_end]
  Delay42/1 -> [start_time]
  Delay43/1 -> [end_time]
  Delay49/1 -> [flag_start_time]
  Delay50/1 -> [flag_end_time]
  pipeline41/1(q) -> wng0/1(scale_16_14)
  pipeline10/1(q) -> [gbe_ip3]
  pipeline11/1(q) -> [gbe_ip2]
  pipeline13/1(q) -> [gbe_ip0]
  Delay126/1 -> [data_enable]
  Delay127/1 -> [sample_mask]
  Delay128/1 -> tvg_spead_time_with_pkt_ctr/1(localtime64)
  Delay129/1 -> tvg_spead_time_with_pkt_ctr/2(data_enable)
  Delay130/1 -> tvg_spead_time_with_pkt_ctr/3(data_mask)
  Delay131/1 -> [tvg_ltime]
  Delay132/1 -> [tvg_stime]
  Delay133/1 -> [tvg_pol0]
  Delay134/1 -> [tvg_pol1]
  Delay105/1 -> bus_convert2/1(din)
  Delay5/1 -> bus_convert3/1(din)
  Delay6/1 -> bus_convert4/1(din)
  Delay9/1 -> bus_convert5/1(din)
  Delay139/1 -> bus_addsub4/1(a)
  Delay7/1 -> bus_addsub5/1(a)
  Delay8/1 -> bus_addsub5/2(b)
  pipeline25/1(q) -> Concat/1
  pipeline26/1(q) -> Concat/2
  pipeline27/1(q) -> Concat1/1
  pipeline28/1(q) -> Concat1/2
  pipeline29/1(q) -> [hdr_0x3101]
  pipeline30/1(q) -> [pol0_id]
  pipeline31/1(q) -> [pol1_id]
  orig_control/1(in_up_cnt_rst) -> pipeline/1(d)
  pipeline/1(q) -> edge_detect3/1(in)
  orig_control/2(in_tvg_select0) -> pipeline1/1(d)
  orig_control/3(in_tvg_select1) -> pipeline2/1(d)
  orig_control/4(in_clr_status) -> pipeline3/1(d)
  orig_control/5(in_gbe_rst) -> pipeline4/1(d)
  orig_control/6(in_gbe_txen) -> pipeline5/1(d)
  orig_control/7(in_msync) -> pipeline6/1(d)
  orig_control/8(in_mrst) -> pipeline7/1(d)
  orig_control/9(in_load_tick_offset) -> pipeline8/1(d)
  pipeline8/1(q) -> edge_detect10/1(in)
  pipeline7/1(q) -> edge_detect2/1(in)
  pipeline6/1(q) -> edge_detect1/1(in)
  pipeline4/1(q) -> Terminator80/1
  pipeline3/1(q) -> edge_detect4/1(in)
  pipeline2/1(q) -> [tvg_select1]
  pipeline1/1(q) -> [tvg_select0]
  pipeline12/1(q) -> [gbe_ip1]
  gbe_iptx0/1(in_reg) -> pipeline13/1(d)
  gbe_iptx1/1(in_reg) -> pipeline12/1(d)
  gbe_iptx2/1(in_reg) -> pipeline11/1(d)
  gbe_iptx3/1(in_reg) -> pipeline10/1(d)
  tick_offset_msw/1(in_reg) -> pipeline17/1(d)
  pipeline17/1(q) -> Concat2/1
  tick_offset_lsw/1(in_reg) -> pipeline18/1(d)
  pipeline18/1(q) -> Concat2/2
  slice1/1 -> pipeline20/1(d)
  pipeline20/1(q) -> local_time_lsw/1(out_reg)
  slice2/1 -> pipeline19/1(d)
  pipeline19/1(q) -> local_time_msw/1(out_reg)
  end_time_lsw/1(in_reg) -> pipeline28/1(d)
  end_time_msw/1(in_reg) -> pipeline27/1(d)
  start_time_lsw/1(in_reg) -> pipeline26/1(d)
  start_time_msw/1(in_reg) -> pipeline25/1(d)
  control_output/4(in_sample_end) -> pipeline24/1(d)
  control_output/3(in_sample_start) -> pipeline23/1(d)
  control_output/2(in_reset_en_time) -> pipeline22/1(d)
  control_output/1(in_load_en_time) -> pipeline21/1(d)
  bus_create/1(bus_out) -> pipeline29/1(d)
  receptor_id/2(in_pol0_id) -> pipeline30/1(d)
  receptor_id/3(in_pol1_id) -> pipeline31/1(d)
  flag_setup/1(in_adc_count) -> pipeline32/1(d)
  flag_setup/2(in_adc_flag) -> pipeline33/1(d)
  flag_setup/3(in_ndiode_flag) -> pipeline34/1(d)
  flag_setup/4(in_load_flags) -> pipeline35/1(d)
  flag_setup/5(in_reset_flags) -> pipeline36/1(d)
  pipeline36/1(q) -> edge_detect8/1(in)
  pipeline35/1(q) -> edge_detect9/1(in)
  pipeline34/1(q) -> [ndiode_flag]
  pipeline33/1(q) -> [adc_flag]
  pipeline32/1(q) -> [adc_count]
  start_flag_msw/1(in_reg) -> pipeline37/1(d)
  pipeline37/1(q) -> Concat4/1
  start_flag_lsw/1(in_reg) -> pipeline38/1(d)
  pipeline38/1(q) -> Concat4/2
  end_flag_msw/1(in_reg) -> pipeline39/1(d)
  pipeline39/1(q) -> Concat5/1
  end_flag_lsw/1(in_reg) -> pipeline40/1(d)
  pipeline40/1(q) -> Concat5/2
  pipeline53/1(q) -> bus_mult1/1(a), [cwg1_tp0]
  pipeline52/1(q) -> bus_mult1/2(b)
  pipeline51/1(q) -> bus_mult/2(b)
  pipeline78/1(q) -> bus_addsub/1(a)
  pipeline79/1(q) -> bus_addsub/2(b)
  pipeline88/1(q) -> bus_addsub1/1(a)
  wng_corr/1(bus_out) -> pipeline88/1(d), pipeline79/1(d)
  pipeline89/1(q) -> bus_addsub1/2(b)
  pipeline91/1(q) -> bus_addsub2/2(b)
  pipeline92/1(q) -> bus_addsub3/1(a)
  pipeline93/1(q) -> bus_addsub3/2(b)
  pipeline94/1(q) -> [cwg_80_0]
  pipeline95/1(q) -> [cwg_80_1]
  Delay2/1 -> bus_addsub4/2(b)
  Delay13/1 -> Logical8/1, Logical6/1
  Delay14/1 -> Logical7/2
  Delay15/1 -> Delay18/1
  Delay16/1 -> Delay19/1
  Delay17/1 -> Logical5/1
  Delay18/1 -> Delay20/1
  Delay19/1 -> Delay21/1
  Delay20/1 -> sample_masking/3(first_samples)
  Delay21/1 -> sample_masking/4(last_samples)
  Delay22/1 -> Logical3/2
  Delay23/1 -> Logical1/1
  Delay24/1 -> Delay25/1
  Delay25/1 -> Delay26/1
  Delay26/1 -> Delay27/1
  Delay27/1 -> sample_masking/1(timei)
  sample_masking/4(flag_valid) -> Delay28/1
  Delay28/1 -> [flag_en]
  Logical1/1 -> sample_masking/7(flag_en)  "flag_en"
  sample_masking/1(timeo) -> Delay29/1
  Delay29/1 -> [masked_time]
  [local_time] -> Delay30/1
  [en_armed] -> Delay31/1
  [local_time] -> Delay32/1, Delay34/1, Delay38/1, Delay40/1
  [start_time] -> Delay33/1
  [end_time] -> Delay35/1, Delay36/1
  Delay30/1 -> Delay24/1
  Delay31/1 -> Delay13/1
  Delay32/1 -> Relational3/1
  Delay33/1 -> Relational3/2
  Delay34/1 -> Relational4/1
  Delay35/1 -> Relational4/2
  Delay36/1 -> Relational5/1
  Delay37/1 -> Relational5/2
  Delay38/1 -> Relational6/1
  Delay39/1 -> Relational6/2
  Delay40/1 -> Relational7/1
  Delay41/1 -> Relational7/2
  Delay44/1 -> Logical4/1, Logical2/1
  Delay45/1 -> Relational/1
  Delay46/1 -> Relational/2
  Delay47/1 -> Relational1/1
  Delay48/1 -> Relational1/2
  Delay51/1 -> Relational2/1
  bus_convert/1(dout) -> [cwg0_tp2], pipeline94/1(d)
  Pulse Generator1/1 -> orig_control/7(sim_7)
  pipeline49/1(q) -> cwg1/1(freq)
  bus_convert2/1(dout) -> [wng0_sum], Delay139/1
  bus_convert3/1(dout) -> [wng1_sum], Delay7/1
  bus_convert4/1(dout) -> Delay2/1
  bus_convert5/1(dout) -> Delay8/1
  bus_convert6/1(dout) -> pipeline50/1(d)
  bus_convert7/1(dout) -> pipeline53/1(d)
  Constant32/1 -> scale_wng1/1(sim_1)
  scale_out0/1(in_scale) -> Gateway Out5/1, pipeline51/1(d)
  pipeline127/1(q) -> Slice6/1
  Slice6/1 -> Convert/1
  Convert/1 -> [pol0_always_on]
  pipeline131/1(q) -> Slice8/1
  Slice8/1 -> Convert2/1
  [pol0_always_on] -> gbe0_traffic_control/1(always_on)
  [pol0_requested_pkts] -> gbe0_traffic_control/2(requested_pkts)
  [pol0_offset_data] -> gbe0_traffic_control/3(offset_data)
  [mrst] -> gbe0_traffic_control/4(mrst)
  [pol0_traffic_trigger] -> gbe0_traffic_control/5(traffic_trigger)
  gbe0_traffic_control/1(gbe_txen_gate) -> [gbe_txen_gate0]
  Constant68/1 -> pol1_sample_offset/1(sim_1)
  pipeline129/1(q) -> [pol1_offset_data]
  Constant67/1 -> pol0_sample_offset/1(sim_1)
  pipeline128/1(q) -> [pol0_offset_data]
  Constant69/1 -> pol0_num_pkts/1(sim_1)
  pipeline126/1(q) -> [pol0_requested_pkts]
  Constant73/1 -> pol1_num_pkts/1(sim_1)
  pipeline134/1(q) -> [pol1_requested_pkts]
  pipeline136/1(q) -> Slice7/1
  Slice7/1 -> Convert1/1
  Convert1/1 -> [pol1_always_on]
  pipeline5/1(q) -> Terminator49/1
  Delay/1 -> pol_traffic_trigger/1(sim_1)
  Constant66/1 -> pol_tx_always_on/1(sim_1)
  Constant77/1 -> pol_tx_always_on/2(sim_2)
  pol0_num_pkts/1(in_pol0_num_pkts) -> pipeline126/1(d)
  pol1_num_pkts/1(in_pol1_num_pkts) -> pipeline134/1(d)
  pol_tx_always_on/1(in_pol0_tx_always_on) -> pipeline127/1(d)
  pol_tx_always_on/2(in_pol1_tx_always_on) -> pipeline136/1(d)
  pol0_sample_offset/1(in_pol0_sample_offset) -> pipeline128/1(d)
  pol1_sample_offset/1(in_pol1_sample_offset) -> pipeline129/1(d)
  Delay52/1 -> pol_traffic_trigger/2(sim_2)
  pol_traffic_trigger/1(in_pol0_tx_trigger) -> pipeline131/1(d)
  pipeline130/1(q) -> Slice9/1
  Slice9/1 -> Convert3/1
  Convert3/1 -> [pol1_traffic_trigger]
  pol_traffic_trigger/2(in_pol1_tx_trigger) -> pipeline130/1(d)
  edge_detect3/1(out) -> Terminator50/1  "mrst"
  Constant64/1 -> freq_cwg0/1(sim_1)
  freq_cwg0/1(in_frequency) -> pipeline45/1(d)
  freq_cwg1/1(in_frequency) -> pipeline49/1(d)
  Constant79/1 -> freq_cwg_corr/1(sim_1)
  freq_cwg_corr/1(in_frequency) -> pipeline47/1(d)
  scale_cwg_corr/1(in_scale) -> pipeline46/1(d)
  AddSub2/1 -> Slice/1
  AddSub1/1 -> Slice1/1
  [tvg_stime] -> AddSub2/1, AddSub1/1
  Constant81/1 -> speadtime0_offset/1(sim_1)
  Slice/1 -> Register5/1
  Slice1/1 -> Register6/1
  speadtime0_offset/1(in_speadtime_offset0) -> AddSub2/2
  Constant82/1 -> speadtime1_offset/1(sim_1)
  speadtime1_offset/1(in_speadtime_offset1) -> AddSub1/2
  [Bus_expand_cwg0] -> CWG_0_Out/1(In1)
  [Bus_expand_cwg1] -> CWG_1_Out/1(In1)
  Convert2/1 -> [pol0_traffic_trigger]
  Constant37/1 -> scale_cwg0/2(sim_2)
  Constant72/1 -> scale_cwg0/1(sim_1)
  Constant41/1 -> scale_cwg1/1(sim_1)
  Constant75/1 -> scale_cwg1/2(sim_2)
  scale_cwg1/1(in_scale) -> Gateway Out18/1, pipeline48/1(d)
  Constant80/1 -> scale_cwg_corr/1(sim_1)
  Constant78/1 -> scale_cwg_corr/2(sim_2)
  Constant58/1 -> scale_out1/1(sim_1)
  Constant63/1 -> scale_out1/2(sim_2)
  scale_out1/2(in_dummy) -> Terminator51/1
  Constant57/1 -> scale_out0/1(sim_1)
  Constant61/1 -> scale_out0/2(sim_2)
  scale_out0/2(in_dummy) -> Terminator/1
  gbe1_traffic_control/1(gbe_txen_gate) -> [gbe_txen_gate1]
  gbe2_traffic_control/1(gbe_txen_gate) -> [gbe_txen_gate2]
  gbe3_traffic_control/1(gbe_txen_gate) -> [gbe_txen_gate3]
  [spead_valid0] -> gbe0_traffic_control/6(spead_valid)
  [pol0_always_on] -> gbe1_traffic_control/1(always_on)
  [pol0_requested_pkts] -> gbe1_traffic_control/2(requested_pkts)
  [pol0_offset_data] -> gbe1_traffic_control/3(offset_data)
  [mrst] -> gbe1_traffic_control/4(mrst)
  [pol0_traffic_trigger] -> gbe1_traffic_control/5(traffic_trigger)
  [pol1_always_on] -> gbe2_traffic_control/1(always_on)
  [pol1_requested_pkts] -> gbe2_traffic_control/2(requested_pkts)
  [pol1_offset_data] -> gbe2_traffic_control/3(offset_data)
  [mrst] -> gbe2_traffic_control/4(mrst)
  [pol1_traffic_trigger] -> gbe2_traffic_control/5(traffic_trigger)
  [pol1_always_on] -> gbe3_traffic_control/1(always_on)
  [pol1_requested_pkts] -> gbe3_traffic_control/2(requested_pkts)
  [pol1_offset_data] -> gbe3_traffic_control/3(offset_data)
  [mrst] -> gbe3_traffic_control/4(mrst)
  [pol1_traffic_trigger] -> gbe3_traffic_control/5(traffic_trigger)
  [spead_valid1] -> gbe1_traffic_control/6(spead_valid)
  [spead_valid2] -> gbe2_traffic_control/6(spead_valid)
  [spead_valid3] -> gbe3_traffic_control/6(spead_valid)
  Constant59/1 -> Delay/1
  Constant40/1 -> Delay52/1
  master_reset_sim7/1 -> dram_addr_offset/1(sim_1)
  master_reset_sim8/1 -> arb_rst/1(sim_1)
  master_reset_sim9/1 -> arb_en/1(sim_1)
  pipeline133/1(q) -> [arb_en0]
  pipeline138/1(q) -> [dram_addr_offset0]
  master_reset_sim1/1 -> dram_read_length/1(sim_1)
  master_reset_sim2/1 -> dram_rd_trigger/1(sim_1)
  pipeline150/1(q) -> [dram_rd_trig0]
  master_reset_sim3/1 -> dram_tvg/1(sim_1)
  master_reset_sim4/1 -> dram_tvg_length/1(sim_1)
  pipeline148/1(q) -> [dram_tvg_length0]
  edge_detect13/1(out) -> [arb_rst0]
  pipeline135/1(q) -> edge_detect13/1(in)
  master_reset_sim5/1 -> dram_rd_repeat/1(sim_1)
  pipeline151/1(q) -> [dram_rd_repeat0]
  pipeline146/1(q) -> Slice13/1, Slice11/1
  Slice13/1 -> Logical17/1, [tvg_sel0]
  Slice11/1 -> Logical17/2
  Logical17/1 -> [dram_tvg0]
  pipeline149/1(q) -> [dram_read_length0]
  master_reset_sim6/1 -> dram_rd_repeat_rate/1(sim_1)
  pipeline137/1(q) -> [dram_rd_repeat_delay0]
  [cwg_80_1] -> pipeline193/1(d)
  [cwg_80_0] -> pipeline190/1(d)
  pipeline158/1(q) -> [source_sel_0]
  pipeline159/1(q) -> [source_sel_1]
  Constant87/1 -> src_sel_cntrl/1(sim_1)
  Constant88/1 -> src_sel_cntrl/2(sim_2)
  src_sel_cntrl/1(in_src_sel_0) -> pipeline158/1(d)
  src_sel_cntrl/2(in_src_sel_1) -> pipeline159/1(d)
  [source_sel_0] -> pipeline189/1(d)
  [source_sel_1] -> pipeline192/1(d)
  Mux5/1 -> pipeline195/1(d)
  Mux4/1 -> pipeline196/1(d)
  master_reset_sim10/1 -> arb_rst/2(sim_2)
  master_reset_sim11/1 -> dram_rd_trigger/2(sim_2)
  master_reset_sim12/1 -> arb_en/2(sim_2)
  dram_rd_repeat_rate/1(in_dram_rd_repeat_rate) -> pipeline137/1(d)
  dram_rd_repeat/1(in_dram_rd_repeat) -> pipeline151/1(d)
  dram_tvg/1(in_arb_tvg) -> pipeline146/1(d)
  dram_tvg_length/1(in_tvg_length) -> pipeline148/1(d)
  dram_addr_offset/1(in_dram_addr_offset) -> pipeline138/1(d)
  dram_read_length/1(in_dram_read_length) -> pipeline149/1(d)
  dram_rd_trigger/1(in_arb_trig) -> pipeline150/1(d)
  dram_rd_trigger/2(in_dummy) -> Terminator55/1
  arb_en/1(in_arb_en) -> pipeline133/1(d)
  arb_en/2(in_dummy) -> Terminator53/1
  arb_rst/1(in_rst) -> pipeline135/1(d)
  arb_rst/2(in_dummy) -> Terminator54/1
  pipeline189/1(q) -> Mux5/1
  pipeline190/1(q) -> Mux5/2
  pipeline191/1(q) -> Mux5/3
  pipeline192/1(q) -> Mux4/1
  pipeline193/1(q) -> Mux4/2
  pipeline194/1(q) -> Mux4/3
  pipeline45/1(q) -> cwg0/1(freq)
  pipeline44/1(q) -> cwg0/2(scale)
  [mrst] -> pipeline180/1(d)
  Constant60/1 -> rpt_en_cwg0/2(sim_2)
  Constant62/1 -> rpt_length_cwg0/1(sim_1)
  rpt_en_cwg0/1(in_en) -> Convert25/1
  rpt_en_cwg0/2(in_dummy) -> Terminator57/1
  Constant70/1 -> rpt_en_cwg0/1(sim_1)
  Convert25/1 -> pipeline181/1(d)
  cwg0/1(bus_out) -> pipeline90/1(d), [Bus_expand_cwg0]
  rpt_length_cwg0/1(in_cwg0_repeat_length) -> pipeline182/1(d)
  pipeline180/1(q) -> cwg0/3(rst)
  pipeline181/1(q) -> cwg0/4(repeat_en)
  pipeline182/1(q) -> cwg0/5(repeat_length)
  pipeline48/1(q) -> cwg1/2(scale)
  Constant76/1 -> rpt_en_cwg1/1(sim_1)
  rpt_en_cwg1/1(in_en) -> Convert26/1
  rpt_en_cwg1/2(in_dummy) -> Terminator59/1
  Constant84/1 -> rpt_en_cwg1/2(sim_2)
  Convert26/1 -> pipeline183/1(d)
  pipeline183/1(q) -> cwg1/4(repeat_en)
  pipeline184/1(q) -> cwg1/5(repeat_length)
  [mrst] -> pipeline185/1(d)
  pipeline185/1(q) -> cwg1/3(rst)
  Constant83/1 -> rpt_length_cwg1/1(sim_1)
  rpt_length_cwg1/1(in_cwg1_repeat_length) -> pipeline184/1(d)
  [adc_count] -> Concat6/1
  Constant90/1 -> Concat6/2
  Delay4/1 -> [status0]
  Delay55/1 -> [status3]
  Delay54/1 -> [status2]
  Delay53/1 -> [status1]
  Concat6/1 -> Delay55/1, Delay4/1, Delay53/1, Delay54/1
  [ndiode_flag] -> Convert28/1
  Logical/1 -> Convert27/1
  Logical19/1 -> Convert30/1
  [adc_flag] -> Convert29/1
  [flag_en] -> Logical/1, Logical19/2
  Convert28/1 -> Logical/2
  Convert29/1 -> Logical19/1
  Convert30/1 -> Concat6/3
  Convert27/1 -> Concat6/4
  cwg0/3(rpt_rst) -> Terminator61/1
  pipeline198/1(q) -> wng0/2(rst)
  Constant23/1 -> man_rst_wng0/1(sim_1)
  Logical20/1 -> pipeline198/1(d)
  man_rst_wng0/1(in_rst) -> [wng0_man_rst], Logical20/2
  Gateway Out13/1 -> To Workspace13/1
  [wng0_rst] -> Logical20/1
  [local_time] -> pipeline203/1(d)
  [mrst] -> pipeline201/1(d)
  [wng0_man_rst] -> pipeline199/1(d)
  wng_rst/1(wng_rst) -> Gateway Out13/1, [wng0_rst]
  Constant89/1 -> rpt_length_wng0/1(sim_1)
  pipeline200/1(q) -> wng_rst/5(num_samples_for_rst)
  pipeline199/1(q) -> wng_rst/4(man_rst)
  pipeline201/1(q) -> wng_rst/3(mrst)
  pipeline202/1(q) -> wng_rst/2(future_time)
  pipeline203/1(q) -> wng_rst/1(local_time)
  Constant95/1 -> rpt_load_time_msw_wng0/1(sim_1)
  Constant93/1 -> rpt_load_time_lsw_wng0/1(sim_1)
  Concat3/1 -> Delay1/1
  pipeline204/1(q) -> Concat3/1
  pipeline205/1(q) -> Concat3/2
  rpt_load_time_lsw_wng0/1(in_reg) -> pipeline205/1(d)
  rpt_load_time_msw_wng0/1(in_reg) -> pipeline204/1(d)
  Delay1/1 -> pipeline202/1(d)
  rpt_length_wng0/1(in_samples) -> pipeline206/1(d)
  pipeline206/1(q) -> pipeline200/1(d)
  [local_time] -> pipeline154/1(d)
  Impulse/1(impulse0) -> [Impulse_gen0]
  pipeline152/1(q) -> Impulse/2(future_time)
  pipeline154/1(q) -> Impulse/1(local_time)
  Constant92/1 -> impulse_load_time_msw/1(sim_1)
  Constant91/1 -> impulse_load_time_lsw/1(sim_1)
  Concat7/1 -> Delay10/1
  pipeline155/1(q) -> Concat7/1
  pipeline160/1(q) -> Concat7/2
  impulse_load_time_lsw/1(in_reg) -> pipeline160/1(d)
  impulse_load_time_msw/1(in_reg) -> pipeline155/1(d)
  Delay10/1 -> pipeline152/1(d)
  pipeline163/1(q) -> Mux5/4
  [Impulse_gen0] -> pipeline163/1(d)
  pipeline164/1(q) -> Mux4/4
  [Impulse_gen0] -> pipeline164/1(d)
  gpio/1 -> Terminator62/1
  Gateway Out/1 -> To Workspace/1
  Impulse/2(impulse_gpio) -> [Impulse_gpio]
  pipeline145/1(q) -> Impulse/3(delay_correction)
  impulse_delay_correction/1(in_reg) -> pipeline145/1(d)
  Constant55/1 -> impulse_delay_correction/1(sim_1)
  pipeline144/1(q) -> Gateway Out/1, gpio/1
  [Impulse_gpio] -> pipeline144/1(d)
  cwg1/3(rpt_rst) -> Terminator60/1
  cwg1/2(dvalid) -> Terminator63/1
  pipeline47/1(q) -> cwg_corr/1(freq)
  pipeline46/1(q) -> cwg_corr/2(scale)
  pipeline147/1(q) -> cwg_corr/3(rst)
  pipeline161/1(q) -> cwg_corr/4(repeat_en)
  pipeline162/1(q) -> cwg_corr/5(repeat_length)
  Constant96/1 -> cwg_corr/6(en)
  [mrst] -> pipeline147/1(d)
  Convert6/1 -> pipeline161/1(d)
  cwg_corr/3(rpt_rst) -> Terminator64/1
  cwg_corr/2(dvalid) -> Terminator65/1
  rpt_en_cwg_corr/1(in_en) -> Convert6/1
  rpt_en_cwg_corr/2(in_dummy) -> Terminator78/1
  Constant97/1 -> rpt_en_cwg_corr/1(sim_1)
  Constant98/1 -> rpt_en_cwg_corr/2(sim_2)
  cwg_corr_repeat_length/1(in_cwg1_repeat_length) -> pipeline162/1(d)
  Constant99/1 -> cwg_corr_repeat_length/1(sim_1)
  [Bus_expand_cwg_corr] -> CWG_1_Out1/1(In1)
  [cwg_80_0] -> CWG_1_Out2/1(In1)
  pipeline50/1(q) -> [cwg0_tp0], bus_mult/1(a)
  [cwg_80_1] -> CWG_1_Out4/1(In1)
  Logical21/1 -> pipeline165/1(d)
  man_rst_wng1/1(in_rst) -> Logical21/2
  [wng0_rst] -> Logical21/1
  Constant100/1 -> man_rst_wng1/1(sim_1)
  Logical24/1 -> pipeline166/1(d)
  man_rst_wng_corr/1(in_rst) -> Logical24/2
  [wng0_rst] -> Logical24/1
  Constant101/1 -> man_rst_wng_corr/1(sim_1)
  Gateway Out3/1 -> To Workspace3/1
  Gateway Out5/1 -> To Workspace5/1
  bus_convert1/1(dout) -> [cwg1_tp2], pipeline95/1(d)
  Gateway Out6/1 -> To Workspace6/1
  Gateway Out17/1 -> To Workspace17/1
  Constant102/1 -> scale_wng1/2(sim_2)
  Constant103/1 -> scale_wng0/2(sim_2)
  Constant104/1 -> pipeline191/1(d)
  Constant105/1 -> pipeline194/1(d)
  [tvg_ltime] -> Delay11/1
  Delay11/1 -> Delay12/1
  [data_80_0] -> Delay56/1
  Delay56/1 -> Delay57/1
  bus_expand14/7(out2) -> pipeline167/1(d)
  bus_expand14/8(lsb_out1) -> pipeline170/1(d)
  bus_expand14/6(out3) -> pipeline171/1(d)
  bus_expand14/5(out4) -> pipeline172/1(d)
  bus_expand14/4(out5) -> pipeline209/1(d)
  bus_expand14/3(out6) -> pipeline210/1(d)
  bus_expand14/2(out7) -> pipeline211/1(d)
  bus_expand14/1(msb_out8) -> pipeline212/1(d)
  pipeline212/1(q) -> ss_fifo_in/1(in_d0)
  pipeline211/1(q) -> ss_fifo_in/2(in_d1)
  pipeline210/1(q) -> ss_fifo_in/3(in_d2)
  pipeline209/1(q) -> ss_fifo_in/4(in_d3)
  pipeline172/1(q) -> ss_fifo_in/5(in_d4)
  pipeline171/1(q) -> ss_fifo_in/6(in_d5)
  pipeline167/1(q) -> ss_fifo_in/7(in_d6)
  pipeline170/1(q) -> ss_fifo_in/8(in_d7)
  Delay57/1 -> bus_expand14/1(bus_in)
  Delay12/1 -> pipeline215/1(d), Relational8/1
  pipeline215/1(q) -> ss_localtime/1(in_time)
  pipeline213/1(q) -> ss_fifo_in/9(in_gpio_trig)
  Delay58/1 -> Delay59/1
  Delay59/1 -> pipeline213/1(d)
  [Impulse_gpio] -> Delay60/1
  Delay60/1 -> Delay58/1
  pipeline214/1(q) -> Impulse/4(Impulse_offset)
  Constant109/1 -> impulse_offset/1(sim_1)
  impulse_offset/1(in_reg) -> pipeline214/1(d)
  Constant108/1 -> ss_trig_time_msw/1(sim_1)
  Constant107/1 -> ss_trig_time_lsw/1(sim_1)
  Concat8/1 -> Delay61/1
  pipeline216/1(q) -> Concat8/1
  pipeline217/1(q) -> Concat8/2
  ss_trig_time_lsw/1(in_reg) -> pipeline217/1(d)
  ss_trig_time_msw/1(in_reg) -> pipeline216/1(d)
  Delay61/1 -> Relational8/2
  Relational8/1 -> edge_detect/1
  pipeline218/1(q) -> ss_fifo_in/10(we)
  [fifoselect] -> pipeline219/1(d), pipeline218/1(d)
  pipeline219/1(q) -> ss_localtime/2(we)
  edge_detect/1 -> ss_fifo_in/11(trig), ss_localtime/3(trig)
  Constant111/1 -> start_load_time_msw/1(sim_1)
  Constant110/1 -> start_load_time_lsw/1(sim_1)
  pipeline220/1(q) -> Concat9/1
  pipeline221/1(q) -> Concat9/2
  start_load_time_msw/1(in_reg) -> pipeline220/1(d)
  start_load_time_lsw/1(in_reg) -> pipeline221/1(d)
  Concat9/1 -> Delay62/1
  Constant113/1 -> stop_load_time_msw/1(sim_1)
  Constant112/1 -> stop_load_time_lsw/1(sim_1)
  pipeline222/1(q) -> Concat10/1
  pipeline223/1(q) -> Concat10/2
  stop_load_time_msw/1(in_reg) -> pipeline222/1(d)
  stop_load_time_lsw/1(in_reg) -> pipeline223/1(d)
  Concat10/1 -> Delay63/1
  Delay62/1 -> pipeline225/1(d)
  Delay63/1 -> pipeline224/1(d)
  pipeline225/1(q) -> Start_stop_Cntrl/1(start_time)
  pipeline224/1(q) -> Start_stop_Cntrl/2(stop_time)
  [mrst] -> Start_stop_Cntrl/3(rst)
  Start_stop_Cntrl/1(Start_Stop_Sel) -> [Start_Stop_Sel]
  pipeline195/1(q) -> Mux3/2
  Mux3/1 -> [data_80_0]
  [Start_Stop_Sel] -> Mux3/1
  Mux6/1 -> [data_80_1]
  pipeline196/1(q) -> Mux6/2
  Constant114/1 -> Mux6/3
  [Start_Stop_Sel] -> Mux6/1
  Constant115/1 -> Mux3/3
  cwg1/1(bus_out) -> pipeline230/1(d)
  Constant74/1 -> cwg1/6(en)
  Constant106/1 -> cwg0/6(en)
  pipeline230/1(q) -> [Bus_expand_cwg1], bus_expand6/1(bus_in), pipeline93/1(d)
  pipeline90/1(q) -> bus_expand2/1(bus_in), bus_addsub2/1(a)
  edge_detect16/1(out) -> pipeline169/1(d)
  control/4(in_cnt_rst) -> edge_detect14/1(in)
  edge_detect14/1(out) -> pipeline143/1(d)
  control/3(in_gbe_rst) -> pipeline173/1(d)
  control/1(in_sys_rst) -> pipeline153/1(d)
  pipeline153/1(q) -> Terminator1/1
  pipeline169/1(q) -> [clr_status]
  pipeline173/1(q) -> [gbe_rst]
  pipeline143/1(q) -> Terminator3/1
  edge_detect15/1(out) -> pipeline156/1(d)
  pipeline156/1(q) -> Terminator2/1
  control/5(in_gbe_cnt_rst) -> edge_detect15/1(in)
  control/2(in_status_clr) -> edge_detect16/1(in)
  [forty_gbe_led_up] -> Delay72/1
  [forty_gbe_led_rx] -> Delay101/1
  [forty_gbe_led_tx] -> Delay110/1
  [forty_gbe_tx_afull] -> Delay107/1
  [forty_gbe_tx_overflow] -> Delay112/1
  [forty_gbe_rx_overrun] -> Delay111/1
  [arb_rst0] -> Terminator9/1
  [arb_en0] -> Terminator10/1
  [dram_rd_repeat0] -> Terminator11/1
  [dram_rd_repeat_delay0] -> Terminator13/1
  [tvg_sel0] -> Terminator14/1
  [dram_tvg0] -> Terminator17/1
  [dram_tvg_length0] -> Terminator19/1
  [dram_addr_offset0] -> Terminator21/1
  [dram_read_length0] -> Terminator22/1
  cwg0/2(dvalid) -> Terminator28/1
  Delay107/1 -> status0/4(out_tx_afull)
  Delay101/1 -> status0/2(out_led_rx)
  Delay112/1 -> status0/5(out_tx_overflow)
  Delay111/1 -> status0/6(out_rx_overrun)
  Delay110/1 -> status0/3(out_led_tx)
  Delay72/1 -> status0/1(out_led_up)
  pipeline15/1(q) -> [gbe_port]
  scale_wng0/1(in_scale) -> Gateway Out17/1, pipeline41/1(d)
  scale_wng1/1(in_scale) -> Gateway Out6/1, pipeline43/1(d)
  pipeline42/1(q) -> wng_corr/1(scale_16_14)
  pipeline166/1(q) -> wng_corr/2(rst)
  pipeline43/1(q) -> wng1/1(scale_16_14)
  pipeline165/1(q) -> wng1/2(rst)
  wng1/1(bus_out) -> [wng1_tp0], pipeline89/1(d)
  Constant65/1 -> freq_cwg1/1(sim_1)
  Constant71/1 -> Terminator29/1
  Constant85/1 -> scale_wng_corr/2(sim_2)
  Gateway Out12/1 -> To Workspace7/1
  scale_wng_corr/1(in_scale) -> Gateway Out12/1, pipeline42/1(d)
  [cwg_80_0] -> Delay76/1
  Delay76/1 -> Delay77/1
  bus_expand1/7(out2) -> pipeline9/1(d)
  bus_expand1/8(lsb_out1) -> pipeline14/1(d)
  bus_expand1/6(out3) -> pipeline16/1(d)
  bus_expand1/5(out4) -> pipeline124/1(d)
  bus_expand1/4(out5) -> pipeline125/1(d)
  bus_expand1/3(out6) -> pipeline139/1(d)
  bus_expand1/2(out7) -> pipeline140/1(d)
  bus_expand1/1(msb_out8) -> pipeline141/1(d)
  pipeline141/1(q) -> ss_cwg0/1(in_d0)
  pipeline140/1(q) -> ss_cwg0/2(in_d1)
  pipeline139/1(q) -> ss_cwg0/3(in_d2)
  pipeline125/1(q) -> ss_cwg0/4(in_d3)
  pipeline124/1(q) -> ss_cwg0/5(in_d4)
  pipeline16/1(q) -> ss_cwg0/6(in_d5)
  pipeline9/1(q) -> ss_cwg0/7(in_d6)
  pipeline14/1(q) -> ss_cwg0/8(in_d7)
  Delay77/1 -> bus_expand1/1(bus_in)
  pipeline142/1(q) -> ss_cwg0/9(in_gpio_trig)
  pipeline157/1(q) -> edge_detect28/1, ss_cwg0/10(we)
  Delay78/1 -> Delay79/1
  [Impulse_gpio] -> Delay78/1
  Delay79/1 -> pipeline142/1(d)
  [fifoselect] -> pipeline157/1(d)
  edge_detect28/1 -> ss_cwg0/11(trig)
  scale_cwg0/1(in_scale) -> Gateway Out16/1, pipeline44/1(d)
  [cwg_80_1] -> Delay85/1
  Delay85/1 -> Delay86/1
  bus_expand5/7(out2) -> pipeline236/1(d)
  bus_expand5/8(lsb_out1) -> pipeline187/1(d)
  bus_expand5/6(out3) -> pipeline235/1(d)
  bus_expand5/5(out4) -> pipeline168/1(d)
  bus_expand5/4(out5) -> pipeline174/1(d)
  bus_expand5/3(out6) -> pipeline186/1(d)
  bus_expand5/2(out7) -> pipeline188/1(d)
  bus_expand5/1(msb_out8) -> pipeline207/1(d)
  pipeline207/1(q) -> ss_cwg1/1(in_d0)
  pipeline188/1(q) -> ss_cwg1/2(in_d1)
  pipeline186/1(q) -> ss_cwg1/3(in_d2)
  pipeline174/1(q) -> ss_cwg1/4(in_d3)
  pipeline168/1(q) -> ss_cwg1/5(in_d4)
  pipeline235/1(q) -> ss_cwg1/6(in_d5)
  pipeline236/1(q) -> ss_cwg1/7(in_d6)
  pipeline187/1(q) -> ss_cwg1/8(in_d7)
  Delay86/1 -> bus_expand5/1(bus_in)
  pipeline233/1(q) -> ss_cwg1/9(in_gpio_trig)
  pipeline234/1(q) -> ss_cwg1/10(we), edge_detect29/1
  Delay115/1 -> Delay116/1
  [Impulse_gpio] -> Delay115/1
  Delay116/1 -> pipeline233/1(d)
  [fifoselect] -> pipeline234/1(d)
  edge_detect29/1 -> ss_cwg1/11(trig)
  Gateway Out16/1 -> To Workspace8/1
  Gateway Out18/1 -> To Workspace10/1
  [gbe_rst] -> forty_gbe/1(rst)
  Constant18/1 -> forty_gbe/7(rx_ack)
  Constant56/1 -> forty_gbe/8(rx_overrun_ack)
  [clr_status] -> forty_gbe/9(debug_rst)
  pipeline258/1(q) -> [forty_gbe_led_up]
  pipeline260/1(q) -> [forty_gbe_led_rx]
  pipeline256/1(q) -> [forty_gbe_led_tx]
  pipeline257/1(q) -> [forty_gbe_tx_afull]
  pipeline259/1(q) -> [forty_gbe_tx_overflow]
  forty_gbe/1(led_up) -> pipeline258/1(d)
  forty_gbe/2(led_rx) -> pipeline260/1(d)
  forty_gbe/3(led_tx) -> pipeline256/1(d)
  forty_gbe/4(tx_afull) -> pipeline257/1(d)
  forty_gbe/5(tx_overflow) -> pipeline259/1(d)
  pipeline261/1(q) -> [forty_gbe_rx_overrun]
  forty_gbe/12(rx_overrun) -> pipeline261/1(d)
  forty_gbe/14(rx_dest_port) -> Terminator30/1
  forty_gbe/13(rx_dest_ip) -> Terminator31/1
  forty_gbe/11(rx_bad_frame) -> Terminator32/1
  forty_gbe/10(rx_end_of_frame) -> Terminator33/1
  forty_gbe/9(rx_source_port) -> Terminator34/1
  forty_gbe/8(rx_source_ip) -> Terminator35/1
  forty_gbe/7(rx_valid) -> Terminator36/1
  forty_gbe/6(rx_data) -> Terminator37/1
  ramp0/1 -> [rampdata0]
  [vld0] -> ramp0/2
  [rdy0] -> ramp0/1
  ramp1/1 -> [rampdata1]
  [vld1] -> ramp1/2
  [rdy1] -> ramp1/1
  speadsnap_control/1(in_speadsnap_arm) -> Delay64/1
  Delay64/1 -> [speadsnap_arm]
  ramp2/1 -> [rampdata2]
  [vld2] -> ramp2/2
  [rdy2] -> ramp2/1
  ramp3/1 -> [rampdata3]
  [vld3] -> ramp3/2
  [rdy3] -> ramp3/1
  Constant116/1 -> gbecontrol/2(sim_2)
  Constant94/1 -> gbecontrol/1(sim_1)
  Constant117/1 -> gbecontrol/3(sim_3)
  Constant118/1 -> gbecontrol/4(sim_4)
  ramp80/1 -> [ramp79]
  [rst_ramp80] -> ramp80/1
  Delay65/1 -> [sel_ramp80]
  test_control/1(in_sel_ramp80) -> Delay65/1
  Delay66/1 -> [rst_ramp80]
  test_control/2(in_rst_ramp80) -> Delay66/1
  [sp256_dv0] -> Mux2/1
  [sp256_data0] -> Mux2/3
  [sp256_data2] -> Mux2/2
  [sp256_dv1] -> pipeline71/1(d)
  Mux2/1 -> Mux7/2
  [sp256_data1] -> pipeline276/1(d)
  [sp256_dv3] -> pipeline72/1(d)
  Mux7/1 -> Mux8/2
  [sp256_data3] -> pipeline277/1(d)
  Mux8/1 -> [sp256_data]
  pipeline276/1(q) -> Mux7/3
  pipeline277/1(q) -> pipeline278/1(d)
  pipeline278/1(q) -> Mux8/3
  [sp256_dvg0] -> Gateway Out15/1, Logical33/1
  [sp256_dvg1] -> Gateway Out19/1, Logical33/2
  [sp256_dvg2] -> Gateway Out20/1, Logical33/3
  [sp256_dvg3] -> Gateway Out21/1, Logical33/4
  Logical33/1 -> pipeline282/1(d)
  pipeline282/1(q) -> pipeline283/1(d)
  pipeline283/1(q) -> Gateway Out2/1, [sp256_dv]
  [sp256_eofg0] -> Gateway Out9/1, Logical10/1
  [sp256_eofg1] -> Gateway Out10/1, Logical10/2
  [sp256_eofg2] -> Gateway Out11/1, Logical10/3
  [sp256_eofg3] -> Gateway Out14/1, Logical10/4
  Logical10/1 -> pipeline284/1(d)
  pipeline284/1(q) -> pipeline70/1(d)
  pipeline70/1(q) -> Gateway Out4/1, [sp256_eof]  "tx_eof"
  [sp256_eof] -> Mux16/1
  Constant139/1 -> Mux16/3
  Constant138/1 -> Mux16/2
  Mux16/1 -> Mux9/3
  Constant137/1 -> Mux9/2
  [sp256_dv] -> Gateway Out1/1, [sp256_dv4], Mux9/1
  [sp256_dv0] -> Mux17/1
  [gbe_ip2] -> Gateway Out24/1, Mux17/2
  [sp256_dv1] -> pipeline54/1(d)
  Mux17/1 -> Mux18/2
  [gbe_ip1] -> Gateway Out23/1, pipeline279/1(d)
  [sp256_dv3] -> pipeline55/1(d)
  Mux18/1 -> Mux19/2
  [gbe_ip3] -> Gateway Out25/1, pipeline280/1(d)
  Mux19/1 -> [gbe_txip]
  pipeline279/1(q) -> Mux18/3
  pipeline280/1(q) -> pipeline281/1(d)
  pipeline281/1(q) -> Mux19/3
  [sp256_dvg0] -> Logical25/1
  [sp256_dvg1] -> Logical22/1
  Logical22/1 -> Logical25/2
  [sp256_dvg3] -> Logical22/3
  [sp256_dvg2] -> Logical22/2
  [sp256_dvg1] -> Logical26/1
  [sp256_dvg0] -> Logical23/1
  Logical23/1 -> Logical26/2
  [sp256_dvg3] -> Logical23/3
  [sp256_dvg2] -> Logical23/2
  [sp256_dvg2] -> Logical28/1
  [sp256_dvg0] -> Logical27/1
  Logical27/1 -> Logical28/2
  [sp256_dvg3] -> Logical27/3
  [sp256_dvg1] -> Logical27/2
  [sp256_dvg3] -> Logical30/1
  [sp256_dvg0] -> Logical29/1
  Logical29/1 -> Logical30/2
  [sp256_dvg2] -> Logical29/3
  [sp256_dvg1] -> Logical29/2
  Logical25/1 -> Logical31/1
  Logical26/1 -> Logical31/2
  Logical28/1 -> Logical31/3
  Logical30/1 -> Logical31/4
  Logical31/1 -> Counter/2  "gbe_dv_error"
  [clr_status] -> Counter/1
  Counter/1 -> gbe_valid_err/1(out_reg)
  pipeline71/1(q) -> Mux7/1
  pipeline72/1(q) -> pipeline73/1(d)
  pipeline73/1(q) -> Mux8/1
  [tvg_select0] -> Delay74/1
  Delay74/1 -> Mux22/1
  Delay75/1 -> Mux22/2
  Delay80/1 -> Mux22/3
  [tvg_pol0] -> Delay75/1
  [data_80_0] -> Delay80/1
  Mux22/1 -> Assert2/1
  [tvg_select1] -> Delay81/1
  Mux23/1 -> Assert3/1  "d80_0"
  [data_80_1] -> Delay83/1
  [tvg_pol1] -> Delay82/1
  Delay81/1 -> Mux23/1
  Delay83/1 -> Mux23/3
  Delay82/1 -> Mux23/2
  Mux9/1 -> Terminator5/1  "tx_dv"
  [gbe_txip] -> Gateway Out8/1
  Gateway Out8/1 -> To Workspace11/1
  Gateway Out9/1 -> To Workspace12/1
  Gateway Out10/1 -> To Workspace14/1
  Gateway Out11/1 -> To Workspace15/1
  Gateway Out14/1 -> To Workspace16/1
  Gateway Out15/1 -> To Workspace18/1
  Gateway Out19/1 -> To Workspace19/1
  Gateway Out20/1 -> To Workspace20/1
  Gateway Out21/1 -> To Workspace21/1
  Gateway Out1/1 -> To Workspace1/1
  Gateway Out2/1 -> To Workspace2/1
  Gateway Out4/1 -> To Workspace4/1
  Gateway Out22/1 -> To Workspace22/1
  Gateway Out23/1 -> To Workspace23/1
  Gateway Out24/1 -> To Workspace24/1
  Gateway Out25/1 -> To Workspace25/1
  [gbe_ip0] -> Gateway Out22/1, Mux17/3
  pipeline54/1(q) -> Mux18/1
  pipeline55/1(q) -> Mux19/1
  Constant/1 -> test_control/1(sim_1)
  Constant21/1 -> test_control/2(sim_2)
  bus_expand/1(msb_out4) -> ?  "tx_d3"
  bus_expand/2(out3) -> ?  "tx_d2"
  bus_expand/3(out2) -> ?  "tx_d1"
  Constant8/1 -> Relational12/2, Relational12/1
  Relational12/1 -> Inverter4/1
  Inverter4/1 -> Logical32/2
  [sp256_eof] -> Logical32/1
  [clr_status] -> Counter1/1
  Counter1/1 -> gbe_last_value_err/1(out_reg)
  Logical32/1 -> Counter1/2  "last_value_error"
  [sp256_data] -> bus_expand/1(bus_in)
  gbecontrol/1(in_gbe0) -> [gbe_txen0]
  gbecontrol/2(in_gbe1) -> [gbe_txen1]
  gbecontrol/3(in_gbe2) -> [gbe_txen2]
  gbecontrol/4(in_gbe3) -> [gbe_txen3]
  [spead_data0] -> spead_snap0/1(in_d64)
  [spead_valid0] -> spead_snap0/2(we)
  [spead_eof0] -> spead_detail/1(in_eof)
  [spead_valid0] -> spead_detail/2(in_we), spead_detail/3(we)
  Logical38/1 -> spead_detail/4(trig), spead_snap0/3(trig)
  [spead_eof0] -> Logical38/2
  [speadsnap_arm] -> Logical38/1
  [sp256_data] -> forty_gbe/2(tx_data)
  [sp256_eof] -> forty_gbe/6(tx_end_of_frame)
  [gbe_txip] -> forty_gbe/4(tx_dest_ip)
  [gbe_port] -> forty_gbe/5(tx_dest_port)
  [clr_status] -> Counter2/1
  Counter2/1 -> tx_afull_cntr/1(out_reg)
  [forty_gbe_tx_afull] -> Counter2/2  "last_value_error"
  [clr_status] -> Counter3/1
  Counter3/1 -> tx_of_cntr/1(out_reg)
  [forty_gbe_tx_overflow] -> Counter3/2  "last_value_error"
  [sp256_dv4] -> forty_gbe/3(tx_valid)
  fifo0/1(fifo_data80) -> pipeline228/1(d)  "data00"
  fifo0/2(fifo_dv) -> pipeline229/1(d)  "dv00"
  fifo0/3(word_start) -> pipeline231/1(d)  "ws00"
  fifo0/4(pkt_start) -> pipeline232/1(d)  "ps00"
  fifo0/5(fifo_full) -> Terminator16/1  "full00"
  fifo0/6(fifo_empty) -> Terminator23/1  "empty00"
  fifo1/1(fifo_data80) -> pipeline100/1(d)  "data01"
  fifo1/2(fifo_dv) -> pipeline101/1(d)  "dv01"
  fifo1/3(word_start) -> pipeline102/1(d)  "ws01"
  fifo1/4(pkt_start) -> pipeline103/1(d)  "ps01"
  pack_80_64_1/2(valid64) -> pipeline116/1(d)  "v64_01"
  pack_80_64_1/1(ready64) -> pipeline115/1(d)  "r64_01"
  fifo1/5(fifo_full) -> Terminator18/1
  fifo1/6(fifo_empty) -> Terminator20/1
  [hdr_0x3101] -> bus_create9/1(in1)
  [pol0_id] -> bus_create9/2(in2)
  [hdr_0x3101] -> bus_create1/1(in1)
  [pol0_id] -> bus_create1/2(in2)
  [speadtime0] -> spead_pack0/8(hdr5_0x1600_DIR), spead_pack0/4(hdr_heap_id)  "timein0"
  bus_create9/1(bus_out) -> spead_pack0/9(hdr6_0x3101_DIR)
  [status0] -> spead_pack0/10(hdr7_0x3102_DIR)
  bus_create1/1(bus_out) -> spead_pack1/9(hdr6_0x3101_DIR)
  [status1] -> spead_pack1/10(hdr7_0x3102_DIR)
  [tvg_ltime] -> fifo_select/1(localtime)
  fifo_select/1(select) -> Delay68/1  "fifo_select"
  Delay68/1 -> fifo0/2(fifo_we_en), [fifoselect], Inverter/1  "fifoselect"
  [speadtime1] -> spead_pack1/4(hdr_heap_id), spead_pack1/8(hdr5_0x1600_DIR)  "timein1"
  pack_80_64_00/1(ready64) -> pipeline112/1(d)  "r64_00"
  pack_80_64_00/2(valid64) -> pipeline113/1(d)  "v64_00"
  [spead_heapsize] -> spead_pack0/5(hdr_heap_size)
  [spead_heapoffset] -> spead_pack0/6(hdr_heap_offset)
  [spead_pktlen] -> spead_pack0/7(hdr_pkt_len_words)
  [spead_heapsize] -> spead_pack1/5(hdr_heap_size)
  [spead_heapoffset] -> spead_pack1/6(hdr_heap_offset)
  [spead_pktlen] -> spead_pack1/7(hdr_pkt_len_words)
  Assert2/1 -> fifo1/1(data80), fifo0/1(data80)
  spead_pack1/4(data_overflow) -> Terminator15/1
  [adc_data_offset] -> spead_pack0/11(hdr8_0x3300)
  [adc_data_offset] -> spead_pack1/11(hdr8_0x3300)
  Constant86/1 -> [spead_heapsize]
  Constant119/1 -> [spead_pktlen]
  Constant120/1 -> [spead_heapoffset]
  spead_pack0/4(data_overflow) -> Terminator12/1
  spead_pack0/3(eof) -> pipeline83/1(d)
  spead_pack0/1(data_out) -> pipeline81/1(d)  "packd"
  spead_pack0/2(valid_out) -> pipeline82/1(d)  "packv"
  spead_pack1/1(data_out) -> pipeline84/1(d)
  spead_pack1/2(valid_out) -> pipeline85/1(d)
  spead_pack1/3(eof) -> pipeline86/1(d)
  Constant131/1 -> [adc_data_offset]
  pipeline81/1(q) -> [spead_data0]
  pipeline82/1(q) -> [spead_valid0]  "sp_dv0"
  pipeline83/1(q) -> [spead_eof0]
  pipeline84/1(q) -> [spead_data1]
  pipeline85/1(q) -> [spead_valid1]  "sp_dv1"
  pipeline86/1(q) -> [spead_eof1]
  pipeline228/1(q) -> Mux12/2  "d80"
  pipeline229/1(q) -> pack_80_64_00/2(valid80)  "v80"
  pipeline231/1(q) -> pack_80_64_00/3(word_start)  "wd_start"
  pipeline232/1(q) -> Delay69/1, pack_80_64_00/4(pkt_start)  "pkt_start"
  pipeline100/1(q) -> Mux13/2
  pipeline101/1(q) -> pack_80_64_1/2(valid80)
  pipeline102/1(q) -> pack_80_64_1/3(word_start)
  pipeline103/1(q) -> Delay70/1, pack_80_64_1/4(pkt_start)
  pipeline112/1(q) -> [rdy0], spead_pack0/1(data64_ready)
  pipeline113/1(q) -> [vld0], spead_pack0/2(data64_valid)
  pipeline115/1(q) -> [rdy1], spead_pack1/1(data64_ready)
  pipeline116/1(q) -> [vld1], spead_pack1/2(data64_valid)
  Inverter/1 -> fifo1/2(fifo_we_en)
  Mux1/1 -> spead_pack0/3(data64)
  Mux20/1 -> spead_pack1/3(data64)
  [spead_data0] -> pipeline57/1(d)
  [spead_valid0] -> pipeline58/1(d)
  wr_addr0/1 -> 64_to_256/1  "waddr"
  [spead_valid0] -> edge_detect27/1(in), edge_detect7/1, pipeline56/1(d)
  Constant122/1 -> 64_to_256/6
  Constant123/1 -> 64_to_256/5
  rd_addr0/1 -> 64_to_256/4, Relational9/2  "rdaddr"
  64_to_256/2 -> pipeline61/1(d)
  edge_detect7/1 -> wr_addr0/1
  pipeline56/1(q) -> wr_addr0/2
  pipeline57/1(q) -> 64_to_256/2
  pipeline58/1(q) -> 64_to_256/3  "dv64_0"
  64_to_256/1 -> Terminator27/1
  edge_detect27/1(out) -> rd_addr0/1, rd_arm/3, rd_arm/1
  Constant130/1 -> Relational9/1
  Relational9/1 -> rd_arm/2  "rd_done"
  rd_arm/1 -> pipeline59/1(d), rd_addr0/2  "rd_en"
  pipeline59/1(q) -> pipeline60/1(d), edge_detect17/1(in)
  edge_detect17/1(out) -> [sp256_eof0]  "eof256_0"
  pipeline61/1(q) -> [sp256_data0]
  fifo2/1(fifo_data80) -> pipeline104/1(d)  "data00"
  fifo2/2(fifo_dv) -> pipeline105/1(d)  "dv00"
  fifo2/3(word_start) -> pipeline106/1(d)  "ws00"
  fifo2/4(pkt_start) -> pipeline107/1(d)  "ps00"
  fifo2/5(fifo_full) -> Terminator8/1  "full00"
  fifo2/6(fifo_empty) -> Terminator26/1  "empty00"
  fifo3/1(fifo_data80) -> pipeline66/1(d)  "data01"
  fifo3/2(fifo_dv) -> pipeline67/1(d)  "dv01"
  fifo3/3(word_start) -> pipeline68/1(d)  "ws01"
  fifo3/4(pkt_start) -> pipeline69/1(d)  "ps01"
  pack_80_64_3/2(valid64) -> pipeline77/1(d)  "v64_01"
  pack_80_64_3/1(ready64) -> pipeline76/1(d)  "r64_01"
  fifo3/5(fifo_full) -> Terminator24/1
  fifo3/6(fifo_empty) -> Terminator25/1
  [hdr_0x3101] -> bus_create3/1(in1)
  [pol1_id] -> bus_create3/2(in2)
  [hdr_0x3101] -> bus_create2/1(in1)
  [pol1_id] -> bus_create2/2(in2)
  [speadtime0] -> spead_pack2/4(hdr_heap_id), spead_pack2/8(hdr5_0x1600_DIR)  "timein0"
  bus_create3/1(bus_out) -> spead_pack2/9(hdr6_0x3101_DIR)
  [status2] -> spead_pack2/10(hdr7_0x3102_DIR)
  bus_create2/1(bus_out) -> spead_pack3/9(hdr6_0x3101_DIR)
  [status3] -> spead_pack3/10(hdr7_0x3102_DIR)
  [tvg_ltime] -> fifo_select1/1(localtime)
  fifo_select1/1(select) -> Delay67/1  "fifo_select"
  Delay67/1 -> Inverter1/1, fifo2/2(fifo_we_en)  "fifoselect"
  [speadtime1] -> spead_pack3/8(hdr5_0x1600_DIR), spead_pack3/4(hdr_heap_id)  "timein1"
  pack_80_64_2/1(ready64) -> pipeline74/1(d)  "r64_00"
  pack_80_64_2/2(valid64) -> pipeline75/1(d)  "v64_00"
  [spead_heapsize] -> spead_pack2/5(hdr_heap_size)
  [spead_heapoffset] -> spead_pack2/6(hdr_heap_offset)
  [spead_pktlen] -> spead_pack2/7(hdr_pkt_len_words)
  [spead_heapsize] -> spead_pack3/5(hdr_heap_size)
  [spead_heapoffset] -> spead_pack3/6(hdr_heap_offset)
  [spead_pktlen] -> spead_pack3/7(hdr_pkt_len_words)
  Assert3/1 -> fifo2/1(data80), fifo3/1(data80)
  spead_pack3/4(data_overflow) -> Terminator7/1
  [adc_data_offset] -> spead_pack2/11(hdr8_0x3300)
  [adc_data_offset] -> spead_pack3/11(hdr8_0x3300)
  spead_pack2/4(data_overflow) -> Terminator4/1
  spead_pack2/3(eof) -> pipeline96/1(d)
  spead_pack2/1(data_out) -> pipeline80/1(d)  "packd"
  spead_pack2/2(valid_out) -> pipeline87/1(d)  "packv"
  spead_pack3/1(data_out) -> pipeline97/1(d)
  spead_pack3/2(valid_out) -> pipeline98/1(d)
  spead_pack3/3(eof) -> pipeline99/1(d)
  pipeline80/1(q) -> [spead_data2]
  pipeline87/1(q) -> [spead_valid2]  "sp_dv0"
  pipeline96/1(q) -> [spead_eof2]
  pipeline97/1(q) -> [spead_data3]
  pipeline98/1(q) -> [spead_valid3]  "sp_dv1"
  pipeline99/1(q) -> [spead_eof3]
  pipeline105/1(q) -> pack_80_64_2/2(valid80)
  pipeline106/1(q) -> pack_80_64_2/3(word_start)
  pipeline107/1(q) -> Delay71/1, pack_80_64_2/4(pkt_start)
  pipeline67/1(q) -> pack_80_64_3/2(valid80)
  pipeline68/1(q) -> pack_80_64_3/3(word_start)
  pipeline69/1(q) -> Delay3/1, pack_80_64_3/4(pkt_start)
  pipeline74/1(q) -> spead_pack2/1(data64_ready), [rdy2]
  pipeline75/1(q) -> spead_pack2/2(data64_valid), [vld2]
  pipeline76/1(q) -> spead_pack3/1(data64_ready), [rdy3]
  pipeline77/1(q) -> spead_pack3/2(data64_valid), [vld3]
  Inverter1/1 -> fifo3/2(fifo_we_en)
  Mux11/1 -> spead_pack3/3(data64)
  [spead_data2] -> pipeline117/1(d)
  [spead_valid2] -> pipeline118/1(d)
  wr_addr2/1 -> 64_to_1/1  "waddr"
  [spead_valid2] -> pipeline114/1(d), edge_detect18/1, edge_detect20/1(in)
  Constant27/1 -> 64_to_1/6
  Constant45/1 -> 64_to_1/5
  rd_addr2/1 -> Relational13/2, 64_to_1/4  "rdaddr"
  64_to_1/2 -> pipeline121/1(d)
  edge_detect18/1 -> wr_addr2/1
  pipeline114/1(q) -> wr_addr2/2
  pipeline117/1(q) -> 64_to_1/2
  pipeline118/1(q) -> 64_to_1/3  "dv64_2"
  64_to_1/1 -> Terminator38/1
  edge_detect20/1(out) -> rd_addr2/1
  Constant121/1 -> Relational13/1
  Relational13/1 -> rd_arm2/2  "rd_done"
  rd_arm2/1 -> rd_addr2/2, pipeline119/1(d)  "rd_en"
  pipeline119/1(q) -> edge_detect19/1(in), pipeline120/1(d)  "dv256"
  edge_detect19/1(out) -> [sp256_eof2]  "eof256_2"
  pipeline120/1(q) -> [sp256_dv2]  "dv256_2"
  pipeline121/1(q) -> [sp256_data2]
  [sp256_eof0] -> rd_arm2/3, rd_arm2/1
  [spead_data1] -> pipeline123/1(d)
  [spead_valid1] -> pipeline132/1(d)
  wr_addr1/1 -> 64_to_2/1  "waddr"
  [spead_valid1] -> pipeline122/1(d), edge_detect21/1, edge_detect23/1(in)
  Constant124/1 -> 64_to_2/6
  Constant125/1 -> 64_to_2/5
  rd_addr1/1 -> Relational10/2, 64_to_2/4  "rdaddr"
  64_to_2/2 -> pipeline177/1(d)
  edge_detect21/1 -> wr_addr1/1
  pipeline122/1(q) -> wr_addr1/2
  pipeline123/1(q) -> 64_to_2/2
  pipeline132/1(q) -> 64_to_2/3  "dv64_1"
  64_to_2/1 -> Terminator39/1
  edge_detect23/1(out) -> rd_arm1/3, rd_arm1/1, rd_addr1/1
  Constant126/1 -> Relational10/1
  Relational10/1 -> rd_arm1/2  "rd_done"
  rd_arm1/1 -> rd_addr1/2, pipeline175/1(d)  "rd_en"
  pipeline175/1(q) -> edge_detect22/1(in), pipeline176/1(d)  "dv256"
  edge_detect22/1(out) -> [sp256_eof1]  "eof256_1"
  pipeline176/1(q) -> [sp256_dv1]  "dv256_1"
  pipeline177/1(q) -> [sp256_data1]
  [spead_data3] -> pipeline179/1(d)
  [spead_valid3] -> pipeline197/1(d)
  wr_addr3/1 -> 64_to_3/1  "waddr"
  [spead_valid3] -> edge_detect26/1(in), edge_detect24/1, pipeline178/1(d)
  Constant127/1 -> 64_to_3/6
  Constant128/1 -> 64_to_3/5
  rd_addr3/1 -> 64_to_3/4, Relational11/2  "rdaddr"
  64_to_3/2 -> pipeline227/1(d)
  edge_detect24/1 -> wr_addr3/1
  pipeline178/1(q) -> wr_addr3/2
  pipeline179/1(q) -> 64_to_3/2
  pipeline197/1(q) -> 64_to_3/3  "dv64_3"
  64_to_3/1 -> Terminator6/1
  edge_detect26/1(out) -> rd_addr3/1
  Constant129/1 -> Relational11/1
  Relational11/1 -> rd_arm3/2  "rd_done"
  rd_arm3/1 -> pipeline208/1(d), rd_addr3/2  "rd_en"
  pipeline208/1(q) -> pipeline226/1(d), edge_detect25/1(in)  "dv256"
  edge_detect25/1(out) -> [sp256_eof3]  "eof256_3"
  pipeline226/1(q) -> [sp256_dv3]  "dv256_3"
  pipeline227/1(q) -> [sp256_data3]
  [sp256_eof1] -> rd_arm3/1, rd_arm3/3
  [gbe_txen0] -> Logical11/2
  pipeline60/1(q) -> [sp256_dv0]  "dv256_0"
  [sp256_eof0] -> Logical11/1
  [sp256_dv0] -> Logical12/1
  [gbe_txen0] -> Logical12/2
  Logical12/1 -> [sp256_dvg0]
  Logical11/1 -> [sp256_eofg0]
  [gbe_txen1] -> Logical13/2
  [sp256_eof1] -> Logical13/1
  [sp256_dv1] -> Logical14/1
  [gbe_txen1] -> Logical14/2
  Logical14/1 -> [sp256_dvg1]
  Logical13/1 -> [sp256_eofg1]
  [gbe_txen2] -> Logical15/2
  [sp256_eof2] -> Logical15/1
  [sp256_dv2] -> Logical16/1
  [gbe_txen2] -> Logical16/2
  Logical16/1 -> [sp256_dvg2]
  Logical15/1 -> [sp256_eofg2]
  [gbe_txen3] -> Logical9/2
  [sp256_eof3] -> Logical9/1
  [sp256_dv3] -> Logical18/1
  [gbe_txen3] -> Logical18/2
  Logical18/1 -> [sp256_dvg3]
  Logical9/1 -> [sp256_eofg3]
  [rampdata0] -> Mux1/2
  [sel_ramp80] -> Mux1/1
  pack_80_64_00/3(data64) -> pipeline108/1(d)
  pipeline108/1(q) -> Mux1/3
  [rampdata1] -> Mux20/2
  [sel_ramp80] -> Mux20/1
  pipeline109/1(q) -> Mux20/3
  pack_80_64_1/3(data64) -> pipeline109/1(d)  "d64_00"
  [rampdata2] -> Mux10/2
  [sel_ramp80] -> Mux10/1
  pipeline110/1(q) -> Mux10/3
  [rampdata3] -> Mux11/2
  [sel_ramp80] -> Mux11/1
  pipeline111/1(q) -> Mux11/3
  pack_80_64_3/3(data64) -> pipeline111/1(d)
  pack_80_64_2/3(data64) -> pipeline110/1(d)
  Mux10/1 -> spead_pack2/3(data64)
  Delay69/1 -> Mux12/1
  [speadtime0] -> Mux12/3
  Mux12/1 -> pack_80_64_00/1(data80)  "d80_in"
  Delay70/1 -> Mux13/1
  [speadtime1] -> Mux13/3
  Mux13/1 -> pack_80_64_1/1(data80)
  Delay71/1 -> Mux14/1
  [speadtime0] -> Mux14/3
  Mux14/1 -> pack_80_64_2/1(data80)
  pipeline104/1(q) -> Mux14/2
  Delay3/1 -> Mux15/1
  [speadtime1] -> Mux15/3
  Mux15/1 -> pack_80_64_3/1(data80)
  pipeline66/1(q) -> Mux15/2
